simulink model "Demo_TISBeamShapes_cs"  (R2014b)
settings: Solver=FixedStepDiscrete  StartTime=0.0  StopTime=0.65  FixedStep=1/20  RelTol=1e-3
PreLoadFcn:
  | mbxruntime.callbacks.PreLoadFcn(bdroot);
  | check_NUTS_defined;
  | 
  | assignin('base',['model_closed_' bdroot],false);
PostLoadFcn:
  | mbxruntime.callbacks.PostLoadFcn(bdroot);
InitFcn:
  | mbxruntime.callbacks.InitFcn(bdroot);
StartFcn:
  | mbxruntime.callbacks.StartFcn(bdroot);
StopFcn:
  | mbxruntime.callbacks.StopFcn(bdroot);
model workspace: external: MAT-File (data not in the file)
undefined symbols (not defined in the file): Demo_TISBeamShapes_cs_011a8b437b9f8e69, Demo_TISBeamShapes_cs_0142ea2f1557d8d7, Demo_TISBeamShapes_cs_017a7d9bca76f440, Demo_TISBeamShapes_cs_024720c4bef5393b, Demo_TISBeamShapes_cs_02ccab9bad151289, Demo_TISBeamShapes_cs_0405f38d677d154d, Demo_TISBeamShapes_cs_04ff6bf95970c620, Demo_TISBeamShapes_cs_053dc575f3a51723, Demo_TISBeamShapes_cs_05aecbce86edff29, Demo_TISBeamShapes_cs_07e5aabef262ff79, Demo_TISBeamShapes_cs_09f6c52f0ff51ce9, Demo_TISBeamShapes_cs_0a8f57eb0b3b3045, Demo_TISBeamShapes_cs_0aa32373a6a68cd2, Demo_TISBeamShapes_cs_0afbbe5f5e24ce0f, Demo_TISBeamShapes_cs_0b39303de350ddcb, Demo_TISBeamShapes_cs_0b9be38c3822ef20, Demo_TISBeamShapes_cs_0c584d0ba0926c34, Demo_TISBeamShapes_cs_0d353a54ded74684, Demo_TISBeamShapes_cs_0e83e05019e43d52, Demo_TISBeamShapes_cs_0f04a582581737c0, Demo_TISBeamShapes_cs_1188b986555cf34f, Demo_TISBeamShapes_cs_11b8ea1198abf687, Demo_TISBeamShapes_cs_11c0571cd6471ba6, Demo_TISBeamShapes_cs_13caba5b40261316, Demo_TISBeamShapes_cs_15569a214ef5cb29, Demo_TISBeamShapes_cs_15f88ebb16dd7ea2, Demo_TISBeamShapes_cs_175a1fcf0f263ce1, Demo_TISBeamShapes_cs_1918ff8c81a32857, Demo_TISBeamShapes_cs_194e8e595a13d2e6, Demo_TISBeamShapes_cs_1a27a7dbb3fbcdbb, Demo_TISBeamShapes_cs_1a494c7f8641a573, Demo_TISBeamShapes_cs_1b017c38f43c5b4b, Demo_TISBeamShapes_cs_1c4cc580bee43225, Demo_TISBeamShapes_cs_1c9c39df8c9251aa, Demo_TISBeamShapes_cs_1d0978b5a4a81629, Demo_TISBeamShapes_cs_1f8d670963c68774, Demo_TISBeamShapes_cs_201dae5c2633ac72, Demo_TISBeamShapes_cs_204926faedc11b3b, Demo_TISBeamShapes_cs_207c04670db5631a, Demo_TISBeamShapes_cs_208dd3dde8789e89, Demo_TISBeamShapes_cs_20cecc5a76828476, Demo_TISBeamShapes_cs_20d64da55f57c800, Demo_TISBeamShapes_cs_21bd21ec0a5e9e24, Demo_TISBeamShapes_cs_21cca4ec9a0489e5, Demo_TISBeamShapes_cs_21d17805a232a810, Demo_TISBeamShapes_cs_22c7f73bd834d507, Demo_TISBeamShapes_cs_22e922ac5e27fa67, Demo_TISBeamShapes_cs_23a17c24d233256c, Demo_TISBeamShapes_cs_23d30f74b2f521d2, Demo_TISBeamShapes_cs_240dd111de20fa52, Demo_TISBeamShapes_cs_244be72567759b92, Demo_TISBeamShapes_cs_2541e0ae6c845c66, Demo_TISBeamShapes_cs_277df13a710d2e6d, Demo_TISBeamShapes_cs_278c9e9dccdcd54f, Demo_TISBeamShapes_cs_28fee81e926d7e28, Demo_TISBeamShapes_cs_29cd51f6b3d7013f, Demo_TISBeamShapes_cs_29d5b88c35ea84dd, Demo_TISBeamShapes_cs_29d910113b92e6ab, Demo_TISBeamShapes_cs_2a48985efc89fc6f, Demo_TISBeamShapes_cs_2b2ff84931628686 ... (+444)
libraries: PreScanSimulinkLibrary x168, PreScanUsefulBlocks x1
(part 1 of 27)
CloseFcn:
  | mbxruntime.callbacks.CloseFcn(bdroot);
  | evalin('base',['clear model_closed_' bdroot]);
settings Model: Creator=PRESCAN  LastModifiedBy=jenkins
settings DataIOCC: SignalLoggingSaveFormat=ModelDataLogs
settings OptimizationCC: InlineParams=on  ExpressionDepthLimit=2147483647  InitFltsAndDblsToZero=on
settings DebuggingCC: SaveWithParameterizedLinksMsg=none  UnderspecifiedInitializationDetection=Classic  MergeDetectMultiDrivingBlocksExec=none  SignalResolutionControl=TryResolveAllWithWarning  SolverPrmCheckMsg=none  MultiTaskDSMMsg=warning  MultiTaskCondExecSysMsg=none  FcnCallInpInsideContextMsg=UseLocalSettings  StateNameClashWarn=warning
settings ModelReferenceCC: UpdateModelReferenceTargets=IfOutOfDate
settings SFSimCC: SimParseCustomCode=off
settings SFSimCC: SimCustomHeaderCode=|
  | #include "prescan.h"
  | #include "prescan_platform.h"
settings RTWCC: IncludeERTFirstTime=on
settings GRTTargetCC: TargetFcnLib=ansi_tfl_tmw.mat  CombineOutputUpdateFcns=off  GRTInterface=on

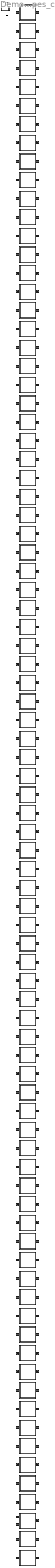
== system Demo_TISBeamShapes_cs ==
  note: Regenerate
  note: Simulink Mode
  note: Open Useful Blocks
  note: 2020.1.0
  note: Version:
  note: Author(s):
  note: N.A.
  note: Descriptive text:
  note: OBU-Beacon ID
  note: Demo Help
  note: This demo illustrates the use of the four possible beam shapes that are available for the TIS. It further illustrates how the TIS output is analyzed in Matlab. Keyword(s) - beamshape - beam - shape
  Cone_1 : Subsystem  Tag=WorldObjectSubSystem  InitFcn=UniqueId = '1098';
      mask init:
      | imagePath=which('Cone.jpg');
      mask Display: image(imread(imagePath));color('white');text(0, 0, ' ID=2\n')
  Controller : Subsystem  Description=8A3CD2955739A82C886C20AE3E253D78460D53180EE2C1B14CC08DF75A70BE77  Priority=-1  LoadFcn=load PreScanControllerData  mask(PreScan Simulation Controller){prescanversion='2020.1.0', ModelReferencing=off, TimeStep=1/20, ControlMode=0, PreScanExecutionMode=on, ControllerCount=0, ControllerIndex=0, ControllerOptions=''}
      mask prompts: prescanversion "PreScan Version"; ModelReferencing "Use Model Referencing"; TimeStep "Upload Period [s]"; ControlMode "Control Mode"; PreScanExecutionMode "Execution Mode"; ControllerCount "Controller Count"; ControllerIndex "Controller Index"; ControllerOptions "Controller Options"
      mask help: Please do not remove this block from the compilation sheet, as it connects the model to the PreScan environment.
      mask init:
      | model = bdroot(gcb);
      | ExperimentFile = mbxruntime.findExperimentFile(model,true); %relative path
      | 
      | [d1, d2, d3, prescandata] = prescan_Settings();
      | ModelDepo = fullfile(prescandata,'ModelDepo'); 
      | 
      | RTmode = mbxruntime.getRTMode(model);
      | 
      | SimulationMode = get_param(bdroot,'SimulationMode');
      | if strcmp(SimulationMode, 'rapid-accelerator')
      |     SimulationMode = 'external';
      | end
      | TargetName = get_param(bdroot,'SystemTargetFile');
      settings: ModelCloseFcn=assignin('base',['model_closed_' bdroot],true);
      mask Help: eval('openHelp(812)')
      mask Display: image(imread('prescanlogo.ico'))
  Cylinder_1 : Subsystem  Tag=WorldObjectSubSystem  InitFcn=UniqueId = '1102';
      mask init:
      | imagePath=which('Cylinder.jpg');
      mask Display: image(imread(imagePath));color('white');text(0, 0, ' ID=1\n')
  Cylinder_2 : Subsystem  Tag=WorldObjectSubSystem  InitFcn=UniqueId = '1103';
      mask init:
      | imagePath=which('Cylinder.jpg');
      mask Display: image(imread(imagePath));color('white');text(0, 0, ' ID=3\n')
  PreScanTerminator : Subsystem  Tag=PreScanTerminator  Priority=999  LoadFcn=load PrescanTerminatorData  mask(PreScan Simulation Terminator){TimeStep=1/20}
      mask prompts: TimeStep "Upload Period [s]"
      mask help: Please do not remove this block from the compilation sheet as it connects the model to the PreScan environment.
      mask Help: eval('openHelp(812)')
      mask Display: image(imread('prescanlogo.ico'))
  SELF_Cone_1 : Subsystem  Tag=sensor/SelfPort  Priority=30  LoadFcn=load('PreScanSelfSensorData.mat')  mask(PreScan Source Block: SELF){}
      mask help: The SELF port shows (state) information of the actor itself. The outputs are position in the experiment's axis system and the GPS coordinates, and the object's absolute velocity and compass heading. For more information, please click Help.
      settings: OpenFcn=open_system([gcb '/Sensor'],'mask')
      mask Help: eval('openHelp(462)')
      mask Display: image(imread('GPS.png'))
  SELF_Cylinder_1 : Subsystem  Tag=sensor/SelfPort  Priority=30  LoadFcn=load('PreScanSelfSensorData.mat')  mask(PreScan Source Block: SELF){}
      mask help: The SELF port shows (state) information of the actor itself. The outputs are position in the experiment's axis system and the GPS coordinates, and the object's absolute velocity and compass heading. For more information, please click Help.
      settings: OpenFcn=open_system([gcb '/Sensor'],'mask')
      mask Help: eval('openHelp(462)')
      mask Display: image(imread('GPS.png'))
  SELF_Cylinder_2 : Subsystem  Tag=sensor/SelfPort  Priority=30  LoadFcn=load('PreScanSelfSensorData.mat')  mask(PreScan Source Block: SELF){}
      mask help: The SELF port shows (state) information of the actor itself. The outputs are position in the experiment's axis system and the GPS coordinates, and the object's absolute velocity and compass heading. For more information, please click Help.
      settings: OpenFcn=open_system([gcb '/Sensor'],'mask')
      mask Help: eval('openHelp(462)')
      mask Display: image(imread('GPS.png'))
  SELF_Sphere_1 : Subsystem  Tag=sensor/SelfPort  Priority=30  LoadFcn=load('PreScanSelfSensorData.mat')  mask(PreScan Source Block: SELF){}
      mask help: The SELF port shows (state) information of the actor itself. The outputs are position in the experiment's axis system and the GPS coordinates, and the object's absolute velocity and compass heading. For more information, please click Help.
      settings: OpenFcn=open_system([gcb '/Sensor'],'mask')
      mask Help: eval('openHelp(462)')
      mask Display: image(imread('GPS.png'))
  SELF_Sphere_10 : Subsystem  Tag=sensor/SelfPort  Priority=30  LoadFcn=load('PreScanSelfSensorData.mat')  mask(PreScan Source Block: SELF){}
      mask help: The SELF port shows (state) information of the actor itself. The outputs are position in the experiment's axis system and the GPS coordinates, and the object's absolute velocity and compass heading. For more information, please click Help.
      settings: OpenFcn=open_system([gcb '/Sensor'],'mask')
      mask Help: eval('openHelp(462)')
      mask Display: image(imread('GPS.png'))
  SELF_Sphere_11 : Subsystem  Tag=sensor/SelfPort  Priority=30  LoadFcn=load('PreScanSelfSensorData.mat')  mask(PreScan Source Block: SELF){}
      mask help: The SELF port shows (state) information of the actor itself. The outputs are position in the experiment's axis system and the GPS coordinates, and the object's absolute velocity and compass heading. For more information, please click Help.
      settings: OpenFcn=open_system([gcb '/Sensor'],'mask')
      mask Help: eval('openHelp(462)')
      mask Display: image(imread('GPS.png'))
  SELF_Sphere_12 : Subsystem  Tag=sensor/SelfPort  Priority=30  LoadFcn=load('PreScanSelfSensorData.mat')  mask(PreScan Source Block: SELF){}
      mask help: The SELF port shows (state) information of the actor itself. The outputs are position in the experiment's axis system and the GPS coordinates, and the object's absolute velocity and compass heading. For more information, please click Help.
      settings: OpenFcn=open_system([gcb '/Sensor'],'mask')
      mask Help: eval('openHelp(462)')
      mask Display: image(imread('GPS.png'))
  SELF_Sphere_13 : Subsystem  Tag=sensor/SelfPort  Priority=30  LoadFcn=load('PreScanSelfSensorData.mat')  mask(PreScan Source Block: SELF){}
      mask help: The SELF port shows (state) information of the actor itself. The outputs are position in the experiment's axis system and the GPS coordinates, and the object's absolute velocity and compass heading. For more information, please click Help.
      settings: OpenFcn=open_system([gcb '/Sensor'],'mask')
      mask Help: eval('openHelp(462)')
      mask Display: image(imread('GPS.png'))
  SELF_Sphere_14 : Subsystem  Tag=sensor/SelfPort  Priority=30  LoadFcn=load('PreScanSelfSensorData.mat')  mask(PreScan Source Block: SELF){}
      mask help: The SELF port shows (state) information of the actor itself. The outputs are position in the experiment's axis system and the GPS coordinates, and the object's absolute velocity and compass heading. For more information, please click Help.
      settings: OpenFcn=open_system([gcb '/Sensor'],'mask')
      mask Help: eval('openHelp(462)')
      mask Display: image(imread('GPS.png'))
  SELF_Sphere_15 : Subsystem  Tag=sensor/SelfPort  Priority=30  LoadFcn=load('PreScanSelfSensorData.mat')  mask(PreScan Source Block: SELF){}
      mask help: The SELF port shows (state) information of the actor itself. The outputs are position in the experiment's axis system and the GPS coordinates, and the object's absolute velocity and compass heading. For more information, please click Help.
      settings: OpenFcn=open_system([gcb '/Sensor'],'mask')
      mask Help: eval('openHelp(462)')
      mask Display: image(imread('GPS.png'))
  SELF_Sphere_16 : Subsystem  Tag=sensor/SelfPort  Priority=30  LoadFcn=load('PreScanSelfSensorData.mat')  mask(PreScan Source Block: SELF){}
      mask help: The SELF port shows (state) information of the actor itself. The outputs are position in the experiment's axis system and the GPS coordinates, and the object's absolute velocity and compass heading. For more information, please click Help.
      settings: OpenFcn=open_system([gcb '/Sensor'],'mask')
      mask Help: eval('openHelp(462)')
      mask Display: image(imread('GPS.png'))
  SELF_Sphere_17 : Subsystem  Tag=sensor/SelfPort  Priority=30  LoadFcn=load('PreScanSelfSensorData.mat')  mask(PreScan Source Block: SELF){}
      mask help: The SELF port shows (state) information of the actor itself. The outputs are position in the experiment's axis system and the GPS coordinates, and the object's absolute velocity and compass heading. For more information, please click Help.
      settings: OpenFcn=open_system([gcb '/Sensor'],'mask')
      mask Help: eval('openHelp(462)')
      mask Display: image(imread('GPS.png'))
  SELF_Sphere_18 : Subsystem  Tag=sensor/SelfPort  Priority=30  LoadFcn=load('PreScanSelfSensorData.mat')  mask(PreScan Source Block: SELF){}
      mask help: The SELF port shows (state) information of the actor itself. The outputs are position in the experiment's axis system and the GPS coordinates, and the object's absolute velocity and compass heading. For more information, please click Help.
      settings: OpenFcn=open_system([gcb '/Sensor'],'mask')
      mask Help: eval('openHelp(462)')
      mask Display: image(imread('GPS.png'))
  SELF_Sphere_19 : Subsystem  Tag=sensor/SelfPort  Priority=30  LoadFcn=load('PreScanSelfSensorData.mat')  mask(PreScan Source Block: SELF){}
      mask help: The SELF port shows (state) information of the actor itself. The outputs are position in the experiment's axis system and the GPS coordinates, and the object's absolute velocity and compass heading. For more information, please click Help.
      settings: OpenFcn=open_system([gcb '/Sensor'],'mask')
      mask Help: eval('openHelp(462)')
      mask Display: image(imread('GPS.png'))
  SELF_Sphere_2 : Subsystem  Tag=sensor/SelfPort  Priority=30  LoadFcn=load('PreScanSelfSensorData.mat')  mask(PreScan Source Block: SELF){}
      mask help: The SELF port shows (state) information of the actor itself. The outputs are position in the experiment's axis system and the GPS coordinates, and the object's absolute velocity and compass heading. For more information, please click Help.
      settings: OpenFcn=open_system([gcb '/Sensor'],'mask')
      mask Help: eval('openHelp(462)')
      mask Display: image(imread('GPS.png'))
  SELF_Sphere_20 : Subsystem  Tag=sensor/SelfPort  Priority=30  LoadFcn=load('PreScanSelfSensorData.mat')  mask(PreScan Source Block: SELF){}
      mask help: The SELF port shows (state) information of the actor itself. The outputs are position in the experiment's axis system and the GPS coordinates, and the object's absolute velocity and compass heading. For more information, please click Help.
      settings: OpenFcn=open_system([gcb '/Sensor'],'mask')
      mask Help: eval('openHelp(462)')
      mask Display: image(imread('GPS.png'))
  SELF_Sphere_21 : Subsystem  Tag=sensor/SelfPort  Priority=30  LoadFcn=load('PreScanSelfSensorData.mat')  mask(PreScan Source Block: SELF){}
      mask help: The SELF port shows (state) information of the actor itself. The outputs are position in the experiment's axis system and the GPS coordinates, and the object's absolute velocity and compass heading. For more information, please click Help.
      settings: OpenFcn=open_system([gcb '/Sensor'],'mask')
      mask Help: eval('openHelp(462)')
      mask Display: image(imread('GPS.png'))
  SELF_Sphere_22 : Subsystem  Tag=sensor/SelfPort  Priority=30  LoadFcn=load('PreScanSelfSensorData.mat')  mask(PreScan Source Block: SELF){}
      mask help: The SELF port shows (state) information of the actor itself. The outputs are position in the experiment's axis system and the GPS coordinates, and the object's absolute velocity and compass heading. For more information, please click Help.
      settings: OpenFcn=open_system([gcb '/Sensor'],'mask')
      mask Help: eval('openHelp(462)')
      mask Display: image(imread('GPS.png'))
  SELF_Sphere_23 : Subsystem  Tag=sensor/SelfPort  Priority=30  LoadFcn=load('PreScanSelfSensorData.mat')  mask(PreScan Source Block: SELF){}
      mask help: The SELF port shows (state) information of the actor itself. The outputs are position in the experiment's axis system and the GPS coordinates, and the object's absolute velocity and compass heading. For more information, please click Help.
      settings: OpenFcn=open_system([gcb '/Sensor'],'mask')
      mask Help: eval('openHelp(462)')
      mask Display: image(imread('GPS.png'))
  SELF_Sphere_24 : Subsystem  Tag=sensor/SelfPort  Priority=30  LoadFcn=load('PreScanSelfSensorData.mat')  mask(PreScan Source Block: SELF){}
      mask help: The SELF port shows (state) information of the actor itself. The outputs are position in the experiment's axis system and the GPS coordinates, and the object's absolute velocity and compass heading. For more information, please click Help.
      settings: OpenFcn=open_system([gcb '/Sensor'],'mask')
      mask Help: eval('openHelp(462)')
      mask Display: image(imread('GPS.png'))
  SELF_Sphere_25 : Subsystem  Tag=sensor/SelfPort  Priority=30  LoadFcn=load('PreScanSelfSensorData.mat')  mask(PreScan Source Block: SELF){}
      mask help: The SELF port shows (state) information of the actor itself. The outputs are position in the experiment's axis system and the GPS coordinates, and the object's absolute velocity and compass heading. For more information, please click Help.
      settings: OpenFcn=open_system([gcb '/Sensor'],'mask')
      mask Help: eval('openHelp(462)')
      mask Display: image(imread('GPS.png'))
  SELF_Sphere_26 : Subsystem  Tag=sensor/SelfPort  Priority=30  LoadFcn=load('PreScanSelfSensorData.mat')  mask(PreScan Source Block: SELF){}
      mask help: The SELF port shows (state) information of the actor itself. The outputs are position in the experiment's axis system and the GPS coordinates, and the object's absolute velocity and compass heading. For more information, please click Help.
      settings: OpenFcn=open_system([gcb '/Sensor'],'mask')
      mask Help: eval('openHelp(462)')
      mask Display: image(imread('GPS.png'))
  SELF_Sphere_27 : Subsystem  Tag=sensor/SelfPort  Priority=30  LoadFcn=load('PreScanSelfSensorData.mat')  mask(PreScan Source Block: SELF){}
      mask help: The SELF port shows (state) information of the actor itself. The outputs are position in the experiment's axis system and the GPS coordinates, and the object's absolute velocity and compass heading. For more information, please click Help.
      settings: OpenFcn=open_system([gcb '/Sensor'],'mask')
      mask Help: eval('openHelp(462)')
      mask Display: image(imread('GPS.png'))
  SELF_Sphere_28 : Subsystem  Tag=sensor/SelfPort  Priority=30  LoadFcn=load('PreScanSelfSensorData.mat')  mask(PreScan Source Block: SELF){}
      mask help: The SELF port shows (state) information of the actor itself. The outputs are position in the experiment's axis system and the GPS coordinates, and the object's absolute velocity and compass heading. For more information, please click Help.
      settings: OpenFcn=open_system([gcb '/Sensor'],'mask')
      mask Help: eval('openHelp(462)')
      mask Display: image(imread('GPS.png'))
  SELF_Sphere_29 : Subsystem  Tag=sensor/SelfPort  Priority=30  LoadFcn=load('PreScanSelfSensorData.mat')  mask(PreScan Source Block: SELF){}
      mask help: The SELF port shows (state) information of the actor itself. The outputs are position in the experiment's axis system and the GPS coordinates, and the object's absolute velocity and compass heading. For more information, please click Help.
      settings: OpenFcn=open_system([gcb '/Sensor'],'mask')
      mask Help: eval('openHelp(462)')
      mask Display: image(imread('GPS.png'))
  SELF_Sphere_3 : Subsystem  Tag=sensor/SelfPort  Priority=30  LoadFcn=load('PreScanSelfSensorData.mat')  mask(PreScan Source Block: SELF){}
      mask help: The SELF port shows (state) information of the actor itself. The outputs are position in the experiment's axis system and the GPS coordinates, and the object's absolute velocity and compass heading. For more information, please click Help.
      settings: OpenFcn=open_system([gcb '/Sensor'],'mask')
      mask Help: eval('openHelp(462)')
      mask Display: image(imread('GPS.png'))
  SELF_Sphere_30 : Subsystem  Tag=sensor/SelfPort  Priority=30  LoadFcn=load('PreScanSelfSensorData.mat')  mask(PreScan Source Block: SELF){}
      mask help: The SELF port shows (state) information of the actor itself. The outputs are position in the experiment's axis system and the GPS coordinates, and the object's absolute velocity and compass heading. For more information, please click Help.
      settings: OpenFcn=open_system([gcb '/Sensor'],'mask')
      mask Help: eval('openHelp(462)')
      mask Display: image(imread('GPS.png'))
  SELF_Sphere_31 : Subsystem  Tag=sensor/SelfPort  Priority=30  LoadFcn=load('PreScanSelfSensorData.mat')  mask(PreScan Source Block: SELF){}
      mask help: The SELF port shows (state) information of the actor itself. The outputs are position in the experiment's axis system and the GPS coordinates, and the object's absolute velocity and compass heading. For more information, please click Help.
      settings: OpenFcn=open_system([gcb '/Sensor'],'mask')
      mask Help: eval('openHelp(462)')
      mask Display: image(imread('GPS.png'))
  SELF_Sphere_32 : Subsystem  Tag=sensor/SelfPort  Priority=30  LoadFcn=load('PreScanSelfSensorData.mat')  mask(PreScan Source Block: SELF){}
      mask help: The SELF port shows (state) information of the actor itself. The outputs are position in the experiment's axis system and the GPS coordinates, and the object's absolute velocity and compass heading. For more information, please click Help.
      settings: OpenFcn=open_system([gcb '/Sensor'],'mask')
      mask Help: eval('openHelp(462)')
      mask Display: image(imread('GPS.png'))
  SELF_Sphere_33 : Subsystem  Tag=sensor/SelfPort  Priority=30  LoadFcn=load('PreScanSelfSensorData.mat')  mask(PreScan Source Block: SELF){}
      mask help: The SELF port shows (state) information of the actor itself. The outputs are position in the experiment's axis system and the GPS coordinates, and the object's absolute velocity and compass heading. For more information, please click Help.
      settings: OpenFcn=open_system([gcb '/Sensor'],'mask')
      mask Help: eval('openHelp(462)')
      mask Display: image(imread('GPS.png'))
  SELF_Sphere_34 : Subsystem  Tag=sensor/SelfPort  Priority=30  LoadFcn=load('PreScanSelfSensorData.mat')  mask(PreScan Source Block: SELF){}
      mask help: The SELF port shows (state) information of the actor itself. The outputs are position in the experiment's axis system and the GPS coordinates, and the object's absolute velocity and compass heading. For more information, please click Help.
      settings: OpenFcn=open_system([gcb '/Sensor'],'mask')
      mask Help: eval('openHelp(462)')
      mask Display: image(imread('GPS.png'))
  SELF_Sphere_35 : Subsystem  Tag=sensor/SelfPort  Priority=30  LoadFcn=load('PreScanSelfSensorData.mat')  mask(PreScan Source Block: SELF){}
      mask help: The SELF port shows (state) information of the actor itself. The outputs are position in the experiment's axis system and the GPS coordinates, and the object's absolute velocity and compass heading. For more information, please click Help.
      settings: OpenFcn=open_system([gcb '/Sensor'],'mask')
      mask Help: eval('openHelp(462)')
      mask Display: image(imread('GPS.png'))
  SELF_Sphere_36 : Subsystem  Tag=sensor/SelfPort  Priority=30  LoadFcn=load('PreScanSelfSensorData.mat')  mask(PreScan Source Block: SELF){}
      mask help: The SELF port shows (state) information of the actor itself. The outputs are position in the experiment's axis system and the GPS coordinates, and the object's absolute velocity and compass heading. For more information, please click Help.
      settings: OpenFcn=open_system([gcb '/Sensor'],'mask')
      mask Help: eval('openHelp(462)')
      mask Display: image(imread('GPS.png'))
  SELF_Sphere_37 : Subsystem  Tag=sensor/SelfPort  Priority=30  LoadFcn=load('PreScanSelfSensorData.mat')  mask(PreScan Source Block: SELF){}
      mask help: The SELF port shows (state) information of the actor itself. The outputs are position in the experiment's axis system and the GPS coordinates, and the object's absolute velocity and compass heading. For more information, please click Help.
      settings: OpenFcn=open_system([gcb '/Sensor'],'mask')
      mask Help: eval('openHelp(462)')
      mask Display: image(imread('GPS.png'))
  SELF_Sphere_38 : Subsystem  Tag=sensor/SelfPort  Priority=30  LoadFcn=load('PreScanSelfSensorData.mat')  mask(PreScan Source Block: SELF){}
      mask help: The SELF port shows (state) information of the actor itself. The outputs are position in the experiment's axis system and the GPS coordinates, and the object's absolute velocity and compass heading. For more information, please click Help.
      settings: OpenFcn=open_system([gcb '/Sensor'],'mask')
      mask Help: eval('openHelp(462)')
      mask Display: image(imread('GPS.png'))
  SELF_Sphere_39 : Subsystem  Tag=sensor/SelfPort  Priority=30  LoadFcn=load('PreScanSelfSensorData.mat')  mask(PreScan Source Block: SELF){}
      mask help: The SELF port shows (state) information of the actor itself. The outputs are position in the experiment's axis system and the GPS coordinates, and the object's absolute velocity and compass heading. For more information, please click Help.
      settings: OpenFcn=open_system([gcb '/Sensor'],'mask')
      mask Help: eval('openHelp(462)')
      mask Display: image(imread('GPS.png'))
  SELF_Sphere_4 : Subsystem  Tag=sensor/SelfPort  Priority=30  LoadFcn=load('PreScanSelfSensorData.mat')  mask(PreScan Source Block: SELF){}
      mask help: The SELF port shows (state) information of the actor itself. The outputs are position in the experiment's axis system and the GPS coordinates, and the object's absolute velocity and compass heading. For more information, please click Help.
      settings: OpenFcn=open_system([gcb '/Sensor'],'mask')
      mask Help: eval('openHelp(462)')
      mask Display: image(imread('GPS.png'))
  SELF_Sphere_40 : Subsystem  Tag=sensor/SelfPort  Priority=30  LoadFcn=load('PreScanSelfSensorData.mat')  mask(PreScan Source Block: SELF){}
      mask help: The SELF port shows (state) information of the actor itself. The outputs are position in the experiment's axis system and the GPS coordinates, and the object's absolute velocity and compass heading. For more information, please click Help.
      settings: OpenFcn=open_system([gcb '/Sensor'],'mask')
      mask Help: eval('openHelp(462)')
      mask Display: image(imread('GPS.png'))
  SELF_Sphere_41 : Subsystem  Tag=sensor/SelfPort  Priority=30  LoadFcn=load('PreScanSelfSensorData.mat')  mask(PreScan Source Block: SELF){}
      mask help: The SELF port shows (state) information of the actor itself. The outputs are position in the experiment's axis system and the GPS coordinates, and the object's absolute velocity and compass heading. For more information, please click Help.
      settings: OpenFcn=open_system([gcb '/Sensor'],'mask')
      mask Help: eval('openHelp(462)')
      mask Display: image(imread('GPS.png'))
  SELF_Sphere_42 : Subsystem  Tag=sensor/SelfPort  Priority=30  LoadFcn=load('PreScanSelfSensorData.mat')  mask(PreScan Source Block: SELF){}
      mask help: The SELF port shows (state) information of the actor itself. The outputs are position in the experiment's axis system and the GPS coordinates, and the object's absolute velocity and compass heading. For more information, please click Help.
      settings: OpenFcn=open_system([gcb '/Sensor'],'mask')
      mask Help: eval('openHelp(462)')
      mask Display: image(imread('GPS.png'))
  SELF_Sphere_43 : Subsystem  Tag=sensor/SelfPort  Priority=30  LoadFcn=load('PreScanSelfSensorData.mat')  mask(PreScan Source Block: SELF){}
      mask help: The SELF port shows (state) information of the actor itself. The outputs are position in the experiment's axis system and the GPS coordinates, and the object's absolute velocity and compass heading. For more information, please click Help.
      settings: OpenFcn=open_system([gcb '/Sensor'],'mask')
      mask Help: eval('openHelp(462)')
      mask Display: image(imread('GPS.png'))
  SELF_Sphere_44 : Subsystem  Tag=sensor/SelfPort  Priority=30  LoadFcn=load('PreScanSelfSensorData.mat')  mask(PreScan Source Block: SELF){}
      mask help: The SELF port shows (state) information of the actor itself. The outputs are position in the experiment's axis system and the GPS coordinates, and the object's absolute velocity and compass heading. For more information, please click Help.
      settings: OpenFcn=open_system([gcb '/Sensor'],'mask')
      mask Help: eval('openHelp(462)')
      mask Display: image(imread('GPS.png'))
  SELF_Sphere_45 : Subsystem  Tag=sensor/SelfPort  Priority=30  LoadFcn=load('PreScanSelfSensorData.mat')  mask(PreScan Source Block: SELF){}
      mask help: The SELF port shows (state) information of the actor itself. The outputs are position in the experiment's axis system and the GPS coordinates, and the object's absolute velocity and compass heading. For more information, please click Help.
      settings: OpenFcn=open_system([gcb '/Sensor'],'mask')
      mask Help: eval('openHelp(462)')
      mask Display: image(imread('GPS.png'))
  SELF_Sphere_46 : Subsystem  Tag=sensor/SelfPort  Priority=30  LoadFcn=load('PreScanSelfSensorData.mat')  mask(PreScan Source Block: SELF){}
      mask help: The SELF port shows (state) information of the actor itself. The outputs are position in the experiment's axis system and the GPS coordinates, and the object's absolute velocity and compass heading. For more information, please click Help.
      settings: OpenFcn=open_system([gcb '/Sensor'],'mask')
      mask Help: eval('openHelp(462)')
      mask Display: image(imread('GPS.png'))
  SELF_Sphere_47 : Subsystem  Tag=sensor/SelfPort  Priority=30  LoadFcn=load('PreScanSelfSensorData.mat')  mask(PreScan Source Block: SELF){}
      mask help: The SELF port shows (state) information of the actor itself. The outputs are position in the experiment's axis system and the GPS coordinates, and the object's absolute velocity and compass heading. For more information, please click Help.
      settings: OpenFcn=open_system([gcb '/Sensor'],'mask')
      mask Help: eval('openHelp(462)')
      mask Display: image(imread('GPS.png'))
  SELF_Sphere_48 : Subsystem  Tag=sensor/SelfPort  Priority=30  LoadFcn=load('PreScanSelfSensorData.mat')  mask(PreScan Source Block: SELF){}
      mask help: The SELF port shows (state) information of the actor itself. The outputs are position in the experiment's axis system and the GPS coordinates, and the object's absolute velocity and compass heading. For more information, please click Help.
      settings: OpenFcn=open_system([gcb '/Sensor'],'mask')
      mask Help: eval('openHelp(462)')
      mask Display: image(imread('GPS.png'))
  SELF_Sphere_49 : Subsystem  Tag=sensor/SelfPort  Priority=30  LoadFcn=load('PreScanSelfSensorData.mat')  mask(PreScan Source Block: SELF){}
      mask help: The SELF port shows (state) information of the actor itself. The outputs are position in the experiment's axis system and the GPS coordinates, and the object's absolute velocity and compass heading. For more information, please click Help.
      settings: OpenFcn=open_system([gcb '/Sensor'],'mask')
      mask Help: eval('openHelp(462)')
      mask Display: image(imread('GPS.png'))
  SELF_Sphere_5 : Subsystem  Tag=sensor/SelfPort  Priority=30  LoadFcn=load('PreScanSelfSensorData.mat')  mask(PreScan Source Block: SELF){}
      mask help: The SELF port shows (state) information of the actor itself. The outputs are position in the experiment's axis system and the GPS coordinates, and the object's absolute velocity and compass heading. For more information, please click Help.
      settings: OpenFcn=open_system([gcb '/Sensor'],'mask')
      mask Help: eval('openHelp(462)')
      mask Display: image(imread('GPS.png'))
  SELF_Sphere_50 : Subsystem  Tag=sensor/SelfPort  Priority=30  LoadFcn=load('PreScanSelfSensorData.mat')  mask(PreScan Source Block: SELF){}
      mask help: The SELF port shows (state) information of the actor itself. The outputs are position in the experiment's axis system and the GPS coordinates, and the object's absolute velocity and compass heading. For more information, please click Help.
      settings: OpenFcn=open_system([gcb '/Sensor'],'mask')
      mask Help: eval('openHelp(462)')
      mask Display: image(imread('GPS.png'))
  SELF_Sphere_51 : Subsystem  Tag=sensor/SelfPort  Priority=30  LoadFcn=load('PreScanSelfSensorData.mat')  mask(PreScan Source Block: SELF){}
      mask help: The SELF port shows (state) information of the actor itself. The outputs are position in the experiment's axis system and the GPS coordinates, and the object's absolute velocity and compass heading. For more information, please click Help.
      settings: OpenFcn=open_system([gcb '/Sensor'],'mask')
      mask Help: eval('openHelp(462)')
      mask Display: image(imread('GPS.png'))
  SELF_Sphere_52 : Subsystem  Tag=sensor/SelfPort  Priority=30  LoadFcn=load('PreScanSelfSensorData.mat')  mask(PreScan Source Block: SELF){}
      mask help: The SELF port shows (state) information of the actor itself. The outputs are position in the experiment's axis system and the GPS coordinates, and the object's absolute velocity and compass heading. For more information, please click Help.
      settings: OpenFcn=open_system([gcb '/Sensor'],'mask')
      mask Help: eval('openHelp(462)')
      mask Display: image(imread('GPS.png'))
  SELF_Sphere_53 : Subsystem  Tag=sensor/SelfPort  Priority=30  LoadFcn=load('PreScanSelfSensorData.mat')  mask(PreScan Source Block: SELF){}
      mask help: The SELF port shows (state) information of the actor itself. The outputs are position in the experiment's axis system and the GPS coordinates, and the object's absolute velocity and compass heading. For more information, please click Help.
      settings: OpenFcn=open_system([gcb '/Sensor'],'mask')
      mask Help: eval('openHelp(462)')
      mask Display: image(imread('GPS.png'))
  SELF_Sphere_54 : Subsystem  Tag=sensor/SelfPort  Priority=30  LoadFcn=load('PreScanSelfSensorData.mat')  mask(PreScan Source Block: SELF){}
      mask help: The SELF port shows (state) information of the actor itself. The outputs are position in the experiment's axis system and the GPS coordinates, and the object's absolute velocity and compass heading. For more information, please click Help.
      settings: OpenFcn=open_system([gcb '/Sensor'],'mask')
      mask Help: eval('openHelp(462)')
      mask Display: image(imread('GPS.png'))
  SELF_Sphere_55 : Subsystem  Tag=sensor/SelfPort  Priority=30  LoadFcn=load('PreScanSelfSensorData.mat')  mask(PreScan Source Block: SELF){}
      mask help: The SELF port shows (state) information of the actor itself. The outputs are position in the experiment's axis system and the GPS coordinates, and the object's absolute velocity and compass heading. For more information, please click Help.
      settings: OpenFcn=open_system([gcb '/Sensor'],'mask')
      mask Help: eval('openHelp(462)')
      mask Display: image(imread('GPS.png'))
  SELF_Sphere_56 : Subsystem  Tag=sensor/SelfPort  Priority=30  LoadFcn=load('PreScanSelfSensorData.mat')  mask(PreScan Source Block: SELF){}
      mask help: The SELF port shows (state) information of the actor itself. The outputs are position in the experiment's axis system and the GPS coordinates, and the object's absolute velocity and compass heading. For more information, please click Help.
      settings: OpenFcn=open_system([gcb '/Sensor'],'mask')
      mask Help: eval('openHelp(462)')
      mask Display: image(imread('GPS.png'))
  SELF_Sphere_57 : Subsystem  Tag=sensor/SelfPort  Priority=30  LoadFcn=load('PreScanSelfSensorData.mat')  mask(PreScan Source Block: SELF){}
      mask help: The SELF port shows (state) information of the actor itself. The outputs are position in the experiment's axis system and the GPS coordinates, and the object's absolute velocity and compass heading. For more information, please click Help.
      settings: OpenFcn=open_system([gcb '/Sensor'],'mask')
      mask Help: eval('openHelp(462)')
      mask Display: image(imread('GPS.png'))
  SELF_Sphere_58 : Subsystem  Tag=sensor/SelfPort  Priority=30  LoadFcn=load('PreScanSelfSensorData.mat')  mask(PreScan Source Block: SELF){}
      mask help: The SELF port shows (state) information of the actor itself. The outputs are position in the experiment's axis system and the GPS coordinates, and the object's absolute velocity and compass heading. For more information, please click Help.
      settings: OpenFcn=open_system([gcb '/Sensor'],'mask')
      mask Help: eval('openHelp(462)')
      mask Display: image(imread('GPS.png'))
  SELF_Sphere_59 : Subsystem  Tag=sensor/SelfPort  Priority=30  LoadFcn=load('PreScanSelfSensorData.mat')  mask(PreScan Source Block: SELF){}
      mask help: The SELF port shows (state) information of the actor itself. The outputs are position in the experiment's axis system and the GPS coordinates, and the object's absolute velocity and compass heading. For more information, please click Help.
      settings: OpenFcn=open_system([gcb '/Sensor'],'mask')
      mask Help: eval('openHelp(462)')
      mask Display: image(imread('GPS.png'))
  SELF_Sphere_6 : Subsystem  Tag=sensor/SelfPort  Priority=30  LoadFcn=load('PreScanSelfSensorData.mat')  mask(PreScan Source Block: SELF){}
      mask help: The SELF port shows (state) information of the actor itself. The outputs are position in the experiment's axis system and the GPS coordinates, and the object's absolute velocity and compass heading. For more information, please click Help.
      settings: OpenFcn=open_system([gcb '/Sensor'],'mask')
      mask Help: eval('openHelp(462)')
      mask Display: image(imread('GPS.png'))
  SELF_Sphere_60 : Subsystem  Tag=sensor/SelfPort  Priority=30  LoadFcn=load('PreScanSelfSensorData.mat')  mask(PreScan Source Block: SELF){}
      mask help: The SELF port shows (state) information of the actor itself. The outputs are position in the experiment's axis system and the GPS coordinates, and the object's absolute velocity and compass heading. For more information, please click Help.
      settings: OpenFcn=open_system([gcb '/Sensor'],'mask')
      mask Help: eval('openHelp(462)')
      mask Display: image(imread('GPS.png'))
  SELF_Sphere_61 : Subsystem  Tag=sensor/SelfPort  Priority=30  LoadFcn=load('PreScanSelfSensorData.mat')  mask(PreScan Source Block: SELF){}
      mask help: The SELF port shows (state) information of the actor itself. The outputs are position in the experiment's axis system and the GPS coordinates, and the object's absolute velocity and compass heading. For more information, please click Help.
      settings: OpenFcn=open_system([gcb '/Sensor'],'mask')
      mask Help: eval('openHelp(462)')
      mask Display: image(imread('GPS.png'))
  SELF_Sphere_62 : Subsystem  Tag=sensor/SelfPort  Priority=30  LoadFcn=load('PreScanSelfSensorData.mat')  mask(PreScan Source Block: SELF){}
      mask help: The SELF port shows (state) information of the actor itself. The outputs are position in the experiment's axis system and the GPS coordinates, and the object's absolute velocity and compass heading. For more information, please click Help.
      settings: OpenFcn=open_system([gcb '/Sensor'],'mask')
      mask Help: eval('openHelp(462)')
      mask Display: image(imread('GPS.png'))
  SELF_Sphere_63 : Subsystem  Tag=sensor/SelfPort  Priority=30  LoadFcn=load('PreScanSelfSensorData.mat')  mask(PreScan Source Block: SELF){}
      mask help: The SELF port shows (state) information of the actor itself. The outputs are position in the experiment's axis system and the GPS coordinates, and the object's absolute velocity and compass heading. For more information, please click Help.
      settings: OpenFcn=open_system([gcb '/Sensor'],'mask')
      mask Help: eval('openHelp(462)')
      mask Display: image(imread('GPS.png'))
  SELF_Sphere_64 : Subsystem  Tag=sensor/SelfPort  Priority=30  LoadFcn=load('PreScanSelfSensorData.mat')  mask(PreScan Source Block: SELF){}
      mask help: The SELF port shows (state) information of the actor itself. The outputs are position in the experiment's axis system and the GPS coordinates, and the object's absolute velocity and compass heading. For more information, please click Help.
      settings: OpenFcn=open_system([gcb '/Sensor'],'mask')
      mask Help: eval('openHelp(462)')
      mask Display: image(imread('GPS.png'))
  SELF_Sphere_65 : Subsystem  Tag=sensor/SelfPort  Priority=30  LoadFcn=load('PreScanSelfSensorData.mat')  mask(PreScan Source Block: SELF){}
      mask help: The SELF port shows (state) information of the actor itself. The outputs are position in the experiment's axis system and the GPS coordinates, and the object's absolute velocity and compass heading. For more information, please click Help.
      settings: OpenFcn=open_system([gcb '/Sensor'],'mask')
      mask Help: eval('openHelp(462)')
      mask Display: image(imread('GPS.png'))
  SELF_Sphere_66 : Subsystem  Tag=sensor/SelfPort  Priority=30  LoadFcn=load('PreScanSelfSensorData.mat')  mask(PreScan Source Block: SELF){}
      mask help: The SELF port shows (state) information of the actor itself. The outputs are position in the experiment's axis system and the GPS coordinates, and the object's absolute velocity and compass heading. For more information, please click Help.
      settings: OpenFcn=open_system([gcb '/Sensor'],'mask')
      mask Help: eval('openHelp(462)')
      mask Display: image(imread('GPS.png'))
  SELF_Sphere_67 : Subsystem  Tag=sensor/SelfPort  Priority=30  LoadFcn=load('PreScanSelfSensorData.mat')  mask(PreScan Source Block: SELF){}
      mask help: The SELF port shows (state) information of the actor itself. The outputs are position in the experiment's axis system and the GPS coordinates, and the object's absolute velocity and compass heading. For more information, please click Help.
      settings: OpenFcn=open_system([gcb '/Sensor'],'mask')
      mask Help: eval('openHelp(462)')
      mask Display: image(imread('GPS.png'))
  SELF_Sphere_68 : Subsystem  Tag=sensor/SelfPort  Priority=30  LoadFcn=load('PreScanSelfSensorData.mat')  mask(PreScan Source Block: SELF){}
      mask help: The SELF port shows (state) information of the actor itself. The outputs are position in the experiment's axis system and the GPS coordinates, and the object's absolute velocity and compass heading. For more information, please click Help.
      settings: OpenFcn=open_system([gcb '/Sensor'],'mask')
      mask Help: eval('openHelp(462)')
      mask Display: image(imread('GPS.png'))
  SELF_Sphere_69 : Subsystem  Tag=sensor/SelfPort  Priority=30  LoadFcn=load('PreScanSelfSensorData.mat')  mask(PreScan Source Block: SELF){}
      mask help: The SELF port shows (state) information of the actor itself. The outputs are position in the experiment's axis system and the GPS coordinates, and the object's absolute velocity and compass heading. For more information, please click Help.
      settings: OpenFcn=open_system([gcb '/Sensor'],'mask')
      mask Help: eval('openHelp(462)')
      mask Display: image(imread('GPS.png'))
  SELF_Sphere_7 : Subsystem  Tag=sensor/SelfPort  Priority=30  LoadFcn=load('PreScanSelfSensorData.mat')  mask(PreScan Source Block: SELF){}
      mask help: The SELF port shows (state) information of the actor itself. The outputs are position in the experiment's axis system and the GPS coordinates, and the object's absolute velocity and compass heading. For more information, please click Help.
      settings: OpenFcn=open_system([gcb '/Sensor'],'mask')
      mask Help: eval('openHelp(462)')
      mask Display: image(imread('GPS.png'))
  SELF_Sphere_70 : Subsystem  Tag=sensor/SelfPort  Priority=30  LoadFcn=load('PreScanSelfSensorData.mat')  mask(PreScan Source Block: SELF){}
      mask help: The SELF port shows (state) information of the actor itself. The outputs are position in the experiment's axis system and the GPS coordinates, and the object's absolute velocity and compass heading. For more information, please click Help.
      settings: OpenFcn=open_system([gcb '/Sensor'],'mask')
      mask Help: eval('openHelp(462)')
      mask Display: image(imread('GPS.png'))
  SELF_Sphere_71 : Subsystem  Tag=sensor/SelfPort  Priority=30  LoadFcn=load('PreScanSelfSensorData.mat')  mask(PreScan Source Block: SELF){}
      mask help: The SELF port shows (state) information of the actor itself. The outputs are position in the experiment's axis system and the GPS coordinates, and the object's absolute velocity and compass heading. For more information, please click Help.
      settings: OpenFcn=open_system([gcb '/Sensor'],'mask')
      mask Help: eval('openHelp(462)')
      mask Display: image(imread('GPS.png'))
  SELF_Sphere_72 : Subsystem  Tag=sensor/SelfPort  Priority=30  LoadFcn=load('PreScanSelfSensorData.mat')  mask(PreScan Source Block: SELF){}
      mask help: The SELF port shows (state) information of the actor itself. The outputs are position in the experiment's axis system and the GPS coordinates, and the object's absolute velocity and compass heading. For more information, please click Help.
      settings: OpenFcn=open_system([gcb '/Sensor'],'mask')
      mask Help: eval('openHelp(462)')
      mask Display: image(imread('GPS.png'))
  SELF_Sphere_73 : Subsystem  Tag=sensor/SelfPort  Priority=30  LoadFcn=load('PreScanSelfSensorData.mat')  mask(PreScan Source Block: SELF){}
      mask help: The SELF port shows (state) information of the actor itself. The outputs are position in the experiment's axis system and the GPS coordinates, and the object's absolute velocity and compass heading. For more information, please click Help.
      settings: OpenFcn=open_system([gcb '/Sensor'],'mask')
      mask Help: eval('openHelp(462)')
      mask Display: image(imread('GPS.png'))
  SELF_Sphere_74 : Subsystem  Tag=sensor/SelfPort  Priority=30  LoadFcn=load('PreScanSelfSensorData.mat')  mask(PreScan Source Block: SELF){}
      mask help: The SELF port shows (state) information of the actor itself. The outputs are position in the experiment's axis system and the GPS coordinates, and the object's absolute velocity and compass heading. For more information, please click Help.
      settings: OpenFcn=open_system([gcb '/Sensor'],'mask')
      mask Help: eval('openHelp(462)')
      mask Display: image(imread('GPS.png'))
  SELF_Sphere_75 : Subsystem  Tag=sensor/SelfPort  Priority=30  LoadFcn=load('PreScanSelfSensorData.mat')  mask(PreScan Source Block: SELF){}
      mask help: The SELF port shows (state) information of the actor itself. The outputs are position in the experiment's axis system and the GPS coordinates, and the object's absolute velocity and compass heading. For more information, please click Help.
      settings: OpenFcn=open_system([gcb '/Sensor'],'mask')
      mask Help: eval('openHelp(462)')
      mask Display: image(imread('GPS.png'))
  SELF_Sphere_76 : Subsystem  Tag=sensor/SelfPort  Priority=30  LoadFcn=load('PreScanSelfSensorData.mat')  mask(PreScan Source Block: SELF){}
      mask help: The SELF port shows (state) information of the actor itself. The outputs are position in the experiment's axis system and the GPS coordinates, and the object's absolute velocity and compass heading. For more information, please click Help.
      settings: OpenFcn=open_system([gcb '/Sensor'],'mask')
      mask Help: eval('openHelp(462)')
      mask Display: image(imread('GPS.png'))
  SELF_Sphere_77 : Subsystem  Tag=sensor/SelfPort  Priority=30  LoadFcn=load('PreScanSelfSensorData.mat')  mask(PreScan Source Block: SELF){}
      mask help: The SELF port shows (state) information of the actor itself. The outputs are position in the experiment's axis system and the GPS coordinates, and the object's absolute velocity and compass heading. For more information, please click Help.
      settings: OpenFcn=open_system([gcb '/Sensor'],'mask')
      mask Help: eval('openHelp(462)')
      mask Display: image(imread('GPS.png'))
  SELF_Sphere_78 : Subsystem  Tag=sensor/SelfPort  Priority=30  LoadFcn=load('PreScanSelfSensorData.mat')  mask(PreScan Source Block: SELF){}
      mask help: The SELF port shows (state) information of the actor itself. The outputs are position in the experiment's axis system and the GPS coordinates, and the object's absolute velocity and compass heading. For more information, please click Help.
      settings: OpenFcn=open_system([gcb '/Sensor'],'mask')
      mask Help: eval('openHelp(462)')
      mask Display: image(imread('GPS.png'))
  SELF_Sphere_79 : Subsystem  Tag=sensor/SelfPort  Priority=30  LoadFcn=load('PreScanSelfSensorData.mat')  mask(PreScan Source Block: SELF){}
      mask help: The SELF port shows (state) information of the actor itself. The outputs are position in the experiment's axis system and the GPS coordinates, and the object's absolute velocity and compass heading. For more information, please click Help.
      settings: OpenFcn=open_system([gcb '/Sensor'],'mask')
      mask Help: eval('openHelp(462)')
      mask Display: image(imread('GPS.png'))
  SELF_Sphere_8 : Subsystem  Tag=sensor/SelfPort  Priority=30  LoadFcn=load('PreScanSelfSensorData.mat')  mask(PreScan Source Block: SELF){}
      mask help: The SELF port shows (state) information of the actor itself. The outputs are position in the experiment's axis system and the GPS coordinates, and the object's absolute velocity and compass heading. For more information, please click Help.
      settings: OpenFcn=open_system([gcb '/Sensor'],'mask')
      mask Help: eval('openHelp(462)')
      mask Display: image(imread('GPS.png'))
  SELF_Sphere_80 : Subsystem  Tag=sensor/SelfPort  Priority=30  LoadFcn=load('PreScanSelfSensorData.mat')  mask(PreScan Source Block: SELF){}
      mask help: The SELF port shows (state) information of the actor itself. The outputs are position in the experiment's axis system and the GPS coordinates, and the object's absolute velocity and compass heading. For more information, please click Help.
      settings: OpenFcn=open_system([gcb '/Sensor'],'mask')
      mask Help: eval('openHelp(462)')
      mask Display: image(imread('GPS.png'))
  SELF_Sphere_81 : Subsystem  Tag=sensor/SelfPort  Priority=30  LoadFcn=load('PreScanSelfSensorData.mat')  mask(PreScan Source Block: SELF){}
      mask help: The SELF port shows (state) information of the actor itself. The outputs are position in the experiment's axis system and the GPS coordinates, and the object's absolute velocity and compass heading. For more information, please click Help.
      settings: OpenFcn=open_system([gcb '/Sensor'],'mask')
      mask Help: eval('openHelp(462)')
      mask Display: image(imread('GPS.png'))
  SELF_Sphere_9 : Subsystem  Tag=sensor/SelfPort  Priority=30  LoadFcn=load('PreScanSelfSensorData.mat')  mask(PreScan Source Block: SELF){}
      mask help: The SELF port shows (state) information of the actor itself. The outputs are position in the experiment's axis system and the GPS coordinates, and the object's absolute velocity and compass heading. For more information, please click Help.
      settings: OpenFcn=open_system([gcb '/Sensor'],'mask')
      mask Help: eval('openHelp(462)')
      mask Display: image(imread('GPS.png'))
  STATE_Cone_1_bus : Subsystem  Tag=actuator/StatePort  Priority=0  LoadFcn=load('PreScanStateActuatorData.mat')  mask(PreScan Sink Block: State){}
      mask help: The Actor State contains a vector signal of size (9x1), containing the following signals: - Position (x,y,z) [m] - Velocity (vx,vy,vz) [m/s] - Angles (Roll, Pitch, Yaw) [rad] The Actor state is defined in the global axis system. The state is superponed on the Initial position defined in the GUI. For more information, please click Help.
      settings: OpenFcn=open_system([gcb '/Actuator'],'mask')
      mask Help: eval('openHelp(222)')
      mask Display: image(imread('State.png'))
  STATE_Cylinder_1_bus : Subsystem  Tag=actuator/StatePort  Priority=0  LoadFcn=load('PreScanStateActuatorData.mat')  mask(PreScan Sink Block: State){}
      mask help: The Actor State contains a vector signal of size (9x1), containing the following signals: - Position (x,y,z) [m] - Velocity (vx,vy,vz) [m/s] - Angles (Roll, Pitch, Yaw) [rad] The Actor state is defined in the global axis system. The state is superponed on the Initial position defined in the GUI. For more information, please click Help.
      settings: OpenFcn=open_system([gcb '/Actuator'],'mask')
      mask Help: eval('openHelp(222)')
      mask Display: image(imread('State.png'))
  STATE_Cylinder_2_bus : Subsystem  Tag=actuator/StatePort  Priority=0  LoadFcn=load('PreScanStateActuatorData.mat')  mask(PreScan Sink Block: State){}
      mask help: The Actor State contains a vector signal of size (9x1), containing the following signals: - Position (x,y,z) [m] - Velocity (vx,vy,vz) [m/s] - Angles (Roll, Pitch, Yaw) [rad] The Actor state is defined in the global axis system. The state is superponed on the Initial position defined in the GUI. For more information, please click Help.
      settings: OpenFcn=open_system([gcb '/Actuator'],'mask')
      mask Help: eval('openHelp(222)')
      mask Display: image(imread('State.png'))
  STATE_Sphere_10_bus : Subsystem  Tag=actuator/StatePort  Priority=0  LoadFcn=load('PreScanStateActuatorData.mat')  mask(PreScan Sink Block: State){}
      mask help: The Actor State contains a vector signal of size (9x1), containing the following signals: - Position (x,y,z) [m] - Velocity (vx,vy,vz) [m/s] - Angles (Roll, Pitch, Yaw) [rad] The Actor state is defined in the global axis system. The state is superponed on the Initial position defined in the GUI. For more information, please click Help.
      settings: OpenFcn=open_system([gcb '/Actuator'],'mask')
      mask Help: eval('openHelp(222)')
      mask Display: image(imread('State.png'))
  STATE_Sphere_11_bus : Subsystem  Tag=actuator/StatePort  Priority=0  LoadFcn=load('PreScanStateActuatorData.mat')  mask(PreScan Sink Block: State){}
      mask help: The Actor State contains a vector signal of size (9x1), containing the following signals: - Position (x,y,z) [m] - Velocity (vx,vy,vz) [m/s] - Angles (Roll, Pitch, Yaw) [rad] The Actor state is defined in the global axis system. The state is superponed on the Initial position defined in the GUI. For more information, please click Help.
      settings: OpenFcn=open_system([gcb '/Actuator'],'mask')
      mask Help: eval('openHelp(222)')
      mask Display: image(imread('State.png'))
  STATE_Sphere_12_bus : Subsystem  Tag=actuator/StatePort  Priority=0  LoadFcn=load('PreScanStateActuatorData.mat')  mask(PreScan Sink Block: State){}
      mask help: The Actor State contains a vector signal of size (9x1), containing the following signals: - Position (x,y,z) [m] - Velocity (vx,vy,vz) [m/s] - Angles (Roll, Pitch, Yaw) [rad] The Actor state is defined in the global axis system. The state is superponed on the Initial position defined in the GUI. For more information, please click Help.
      settings: OpenFcn=open_system([gcb '/Actuator'],'mask')
      mask Help: eval('openHelp(222)')
      mask Display: image(imread('State.png'))
  STATE_Sphere_13_bus : Subsystem  Tag=actuator/StatePort  Priority=0  LoadFcn=load('PreScanStateActuatorData.mat')  mask(PreScan Sink Block: State){}
      mask help: The Actor State contains a vector signal of size (9x1), containing the following signals: - Position (x,y,z) [m] - Velocity (vx,vy,vz) [m/s] - Angles (Roll, Pitch, Yaw) [rad] The Actor state is defined in the global axis system. The state is superponed on the Initial position defined in the GUI. For more information, please click Help.
      settings: OpenFcn=open_system([gcb '/Actuator'],'mask')
      mask Help: eval('openHelp(222)')
      mask Display: image(imread('State.png'))
  STATE_Sphere_14_bus : Subsystem  Tag=actuator/StatePort  Priority=0  LoadFcn=load('PreScanStateActuatorData.mat')  mask(PreScan Sink Block: State){}
      mask help: The Actor State contains a vector signal of size (9x1), containing the following signals: - Position (x,y,z) [m] - Velocity (vx,vy,vz) [m/s] - Angles (Roll, Pitch, Yaw) [rad] The Actor state is defined in the global axis system. The state is superponed on the Initial position defined in the GUI. For more information, please click Help.
      settings: OpenFcn=open_system([gcb '/Actuator'],'mask')
      mask Help: eval('openHelp(222)')
      mask Display: image(imread('State.png'))
  STATE_Sphere_15_bus : Subsystem  Tag=actuator/StatePort  Priority=0  LoadFcn=load('PreScanStateActuatorData.mat')  mask(PreScan Sink Block: State){}
      mask help: The Actor State contains a vector signal of size (9x1), containing the following signals: - Position (x,y,z) [m] - Velocity (vx,vy,vz) [m/s] - Angles (Roll, Pitch, Yaw) [rad] The Actor state is defined in the global axis system. The state is superponed on the Initial position defined in the GUI. For more information, please click Help.
      settings: OpenFcn=open_system([gcb '/Actuator'],'mask')
      mask Help: eval('openHelp(222)')
      mask Display: image(imread('State.png'))
  STATE_Sphere_16_bus : Subsystem  Tag=actuator/StatePort  Priority=0  LoadFcn=load('PreScanStateActuatorData.mat')  mask(PreScan Sink Block: State){}
      mask help: The Actor State contains a vector signal of size (9x1), containing the following signals: - Position (x,y,z) [m] - Velocity (vx,vy,vz) [m/s] - Angles (Roll, Pitch, Yaw) [rad] The Actor state is defined in the global axis system. The state is superponed on the Initial position defined in the GUI. For more information, please click Help.
      settings: OpenFcn=open_system([gcb '/Actuator'],'mask')
      mask Help: eval('openHelp(222)')
      mask Display: image(imread('State.png'))
  STATE_Sphere_17_bus : Subsystem  Tag=actuator/StatePort  Priority=0  LoadFcn=load('PreScanStateActuatorData.mat')  mask(PreScan Sink Block: State){}
      mask help: The Actor State contains a vector signal of size (9x1), containing the following signals: - Position (x,y,z) [m] - Velocity (vx,vy,vz) [m/s] - Angles (Roll, Pitch, Yaw) [rad] The Actor state is defined in the global axis system. The state is superponed on the Initial position defined in the GUI. For more information, please click Help.
      settings: OpenFcn=open_system([gcb '/Actuator'],'mask')
      mask Help: eval('openHelp(222)')
      mask Display: image(imread('State.png'))
  STATE_Sphere_18_bus : Subsystem  Tag=actuator/StatePort  Priority=0  LoadFcn=load('PreScanStateActuatorData.mat')  mask(PreScan Sink Block: State){}
      mask help: The Actor State contains a vector signal of size (9x1), containing the following signals: - Position (x,y,z) [m] - Velocity (vx,vy,vz) [m/s] - Angles (Roll, Pitch, Yaw) [rad] The Actor state is defined in the global axis system. The state is superponed on the Initial position defined in the GUI. For more information, please click Help.
      settings: OpenFcn=open_system([gcb '/Actuator'],'mask')
      mask Help: eval('openHelp(222)')
      mask Display: image(imread('State.png'))
  STATE_Sphere_19_bus : Subsystem  Tag=actuator/StatePort  Priority=0  LoadFcn=load('PreScanStateActuatorData.mat')  mask(PreScan Sink Block: State){}
      mask help: The Actor State contains a vector signal of size (9x1), containing the following signals: - Position (x,y,z) [m] - Velocity (vx,vy,vz) [m/s] - Angles (Roll, Pitch, Yaw) [rad] The Actor state is defined in the global axis system. The state is superponed on the Initial position defined in the GUI. For more information, please click Help.
      settings: OpenFcn=open_system([gcb '/Actuator'],'mask')
      mask Help: eval('openHelp(222)')
      mask Display: image(imread('State.png'))
  STATE_Sphere_1_bus : Subsystem  Tag=actuator/StatePort  Priority=0  LoadFcn=load('PreScanStateActuatorData.mat')  mask(PreScan Sink Block: State){}
      mask help: The Actor State contains a vector signal of size (9x1), containing the following signals: - Position (x,y,z) [m] - Velocity (vx,vy,vz) [m/s] - Angles (Roll, Pitch, Yaw) [rad] The Actor state is defined in the global axis system. The state is superponed on the Initial position defined in the GUI. For more information, please click Help.
      settings: OpenFcn=open_system([gcb '/Actuator'],'mask')
      mask Help: eval('openHelp(222)')
      mask Display: image(imread('State.png'))
  STATE_Sphere_20_bus : Subsystem  Tag=actuator/StatePort  Priority=0  LoadFcn=load('PreScanStateActuatorData.mat')  mask(PreScan Sink Block: State){}
      mask help: The Actor State contains a vector signal of size (9x1), containing the following signals: - Position (x,y,z) [m] - Velocity (vx,vy,vz) [m/s] - Angles (Roll, Pitch, Yaw) [rad] The Actor state is defined in the global axis system. The state is superponed on the Initial position defined in the GUI. For more information, please click Help.
      settings: OpenFcn=open_system([gcb '/Actuator'],'mask')
      mask Help: eval('openHelp(222)')
      mask Display: image(imread('State.png'))
  STATE_Sphere_21_bus : Subsystem  Tag=actuator/StatePort  Priority=0  LoadFcn=load('PreScanStateActuatorData.mat')  mask(PreScan Sink Block: State){}
      mask help: The Actor State contains a vector signal of size (9x1), containing the following signals: - Position (x,y,z) [m] - Velocity (vx,vy,vz) [m/s] - Angles (Roll, Pitch, Yaw) [rad] The Actor state is defined in the global axis system. The state is superponed on the Initial position defined in the GUI. For more information, please click Help.
      settings: OpenFcn=open_system([gcb '/Actuator'],'mask')
      mask Help: eval('openHelp(222)')
      mask Display: image(imread('State.png'))
  STATE_Sphere_22_bus : Subsystem  Tag=actuator/StatePort  Priority=0  LoadFcn=load('PreScanStateActuatorData.mat')  mask(PreScan Sink Block: State){}
      mask help: The Actor State contains a vector signal of size (9x1), containing the following signals: - Position (x,y,z) [m] - Velocity (vx,vy,vz) [m/s] - Angles (Roll, Pitch, Yaw) [rad] The Actor state is defined in the global axis system. The state is superponed on the Initial position defined in the GUI. For more information, please click Help.
      settings: OpenFcn=open_system([gcb '/Actuator'],'mask')
      mask Help: eval('openHelp(222)')
      mask Display: image(imread('State.png'))
  STATE_Sphere_23_bus : Subsystem  Tag=actuator/StatePort  Priority=0  LoadFcn=load('PreScanStateActuatorData.mat')  mask(PreScan Sink Block: State){}
      mask help: The Actor State contains a vector signal of size (9x1), containing the following signals: - Position (x,y,z) [m] - Velocity (vx,vy,vz) [m/s] - Angles (Roll, Pitch, Yaw) [rad] The Actor state is defined in the global axis system. The state is superponed on the Initial position defined in the GUI. For more information, please click Help.
      settings: OpenFcn=open_system([gcb '/Actuator'],'mask')
      mask Help: eval('openHelp(222)')
      mask Display: image(imread('State.png'))
  STATE_Sphere_24_bus : Subsystem  Tag=actuator/StatePort  Priority=0  LoadFcn=load('PreScanStateActuatorData.mat')  mask(PreScan Sink Block: State){}
      mask help: The Actor State contains a vector signal of size (9x1), containing the following signals: - Position (x,y,z) [m] - Velocity (vx,vy,vz) [m/s] - Angles (Roll, Pitch, Yaw) [rad] The Actor state is defined in the global axis system. The state is superponed on the Initial position defined in the GUI. For more information, please click Help.
      settings: OpenFcn=open_system([gcb '/Actuator'],'mask')
      mask Help: eval('openHelp(222)')
      mask Display: image(imread('State.png'))
  STATE_Sphere_25_bus : Subsystem  Tag=actuator/StatePort  Priority=0  LoadFcn=load('PreScanStateActuatorData.mat')  mask(PreScan Sink Block: State){}
      mask help: The Actor State contains a vector signal of size (9x1), containing the following signals: - Position (x,y,z) [m] - Velocity (vx,vy,vz) [m/s] - Angles (Roll, Pitch, Yaw) [rad] The Actor state is defined in the global axis system. The state is superponed on the Initial position defined in the GUI. For more information, please click Help.
      settings: OpenFcn=open_system([gcb '/Actuator'],'mask')
      mask Help: eval('openHelp(222)')
      mask Display: image(imread('State.png'))
  STATE_Sphere_26_bus : Subsystem  Tag=actuator/StatePort  Priority=0  LoadFcn=load('PreScanStateActuatorData.mat')  mask(PreScan Sink Block: State){}
      mask help: The Actor State contains a vector signal of size (9x1), containing the following signals: - Position (x,y,z) [m] - Velocity (vx,vy,vz) [m/s] - Angles (Roll, Pitch, Yaw) [rad] The Actor state is defined in the global axis system. The state is superponed on the Initial position defined in the GUI. For more information, please click Help.
      settings: OpenFcn=open_system([gcb '/Actuator'],'mask')
      mask Help: eval('openHelp(222)')
      mask Display: image(imread('State.png'))
  STATE_Sphere_27_bus : Subsystem  Tag=actuator/StatePort  Priority=0  LoadFcn=load('PreScanStateActuatorData.mat')  mask(PreScan Sink Block: State){}
      mask help: The Actor State contains a vector signal of size (9x1), containing the following signals: - Position (x,y,z) [m] - Velocity (vx,vy,vz) [m/s] - Angles (Roll, Pitch, Yaw) [rad] The Actor state is defined in the global axis system. The state is superponed on the Initial position defined in the GUI. For more information, please click Help.
      settings: OpenFcn=open_system([gcb '/Actuator'],'mask')
      mask Help: eval('openHelp(222)')
      mask Display: image(imread('State.png'))
  STATE_Sphere_28_bus : Subsystem  Tag=actuator/StatePort  Priority=0  LoadFcn=load('PreScanStateActuatorData.mat')  mask(PreScan Sink Block: State){}
      mask help: The Actor State contains a vector signal of size (9x1), containing the following signals: - Position (x,y,z) [m] - Velocity (vx,vy,vz) [m/s] - Angles (Roll, Pitch, Yaw) [rad] The Actor state is defined in the global axis system. The state is superponed on the Initial position defined in the GUI. For more information, please click Help.
      settings: OpenFcn=open_system([gcb '/Actuator'],'mask')
      mask Help: eval('openHelp(222)')
      mask Display: image(imread('State.png'))
  STATE_Sphere_29_bus : Subsystem  Tag=actuator/StatePort  Priority=0  LoadFcn=load('PreScanStateActuatorData.mat')  mask(PreScan Sink Block: State){}
      mask help: The Actor State contains a vector signal of size (9x1), containing the following signals: - Position (x,y,z) [m] - Velocity (vx,vy,vz) [m/s] - Angles (Roll, Pitch, Yaw) [rad] The Actor state is defined in the global axis system. The state is superponed on the Initial position defined in the GUI. For more information, please click Help.
      settings: OpenFcn=open_system([gcb '/Actuator'],'mask')
      mask Help: eval('openHelp(222)')
      mask Display: image(imread('State.png'))
  STATE_Sphere_2_bus : Subsystem  Tag=actuator/StatePort  Priority=0  LoadFcn=load('PreScanStateActuatorData.mat')  mask(PreScan Sink Block: State){}
      mask help: The Actor State contains a vector signal of size (9x1), containing the following signals: - Position (x,y,z) [m] - Velocity (vx,vy,vz) [m/s] - Angles (Roll, Pitch, Yaw) [rad] The Actor state is defined in the global axis system. The state is superponed on the Initial position defined in the GUI. For more information, please click Help.
      settings: OpenFcn=open_system([gcb '/Actuator'],'mask')
      mask Help: eval('openHelp(222)')
      mask Display: image(imread('State.png'))
  STATE_Sphere_30_bus : Subsystem  Tag=actuator/StatePort  Priority=0  LoadFcn=load('PreScanStateActuatorData.mat')  mask(PreScan Sink Block: State){}
      mask help: The Actor State contains a vector signal of size (9x1), containing the following signals: - Position (x,y,z) [m] - Velocity (vx,vy,vz) [m/s] - Angles (Roll, Pitch, Yaw) [rad] The Actor state is defined in the global axis system. The state is superponed on the Initial position defined in the GUI. For more information, please click Help.
      settings: OpenFcn=open_system([gcb '/Actuator'],'mask')
      mask Help: eval('openHelp(222)')
      mask Display: image(imread('State.png'))
  STATE_Sphere_31_bus : Subsystem  Tag=actuator/StatePort  Priority=0  LoadFcn=load('PreScanStateActuatorData.mat')  mask(PreScan Sink Block: State){}
      mask help: The Actor State contains a vector signal of size (9x1), containing the following signals: - Position (x,y,z) [m] - Velocity (vx,vy,vz) [m/s] - Angles (Roll, Pitch, Yaw) [rad] The Actor state is defined in the global axis system. The state is superponed on the Initial position defined in the GUI. For more information, please click Help.
      settings: OpenFcn=open_system([gcb '/Actuator'],'mask')
      mask Help: eval('openHelp(222)')
      mask Display: image(imread('State.png'))
  STATE_Sphere_32_bus : Subsystem  Tag=actuator/StatePort  Priority=0  LoadFcn=load('PreScanStateActuatorData.mat')  mask(PreScan Sink Block: State){}
      mask help: The Actor State contains a vector signal of size (9x1), containing the following signals: - Position (x,y,z) [m] - Velocity (vx,vy,vz) [m/s] - Angles (Roll, Pitch, Yaw) [rad] The Actor state is defined in the global axis system. The state is superponed on the Initial position defined in the GUI. For more information, please click Help.
      settings: OpenFcn=open_system([gcb '/Actuator'],'mask')
      mask Help: eval('openHelp(222)')
      mask Display: image(imread('State.png'))
  STATE_Sphere_33_bus : Subsystem  Tag=actuator/StatePort  Priority=0  LoadFcn=load('PreScanStateActuatorData.mat')  mask(PreScan Sink Block: State){}
      mask help: The Actor State contains a vector signal of size (9x1), containing the following signals: - Position (x,y,z) [m] - Velocity (vx,vy,vz) [m/s] - Angles (Roll, Pitch, Yaw) [rad] The Actor state is defined in the global axis system. The state is superponed on the Initial position defined in the GUI. For more information, please click Help.
      settings: OpenFcn=open_system([gcb '/Actuator'],'mask')
      mask Help: eval('openHelp(222)')
      mask Display: image(imread('State.png'))
  STATE_Sphere_34_bus : Subsystem  Tag=actuator/StatePort  Priority=0  LoadFcn=load('PreScanStateActuatorData.mat')  mask(PreScan Sink Block: State){}
      mask help: The Actor State contains a vector signal of size (9x1), containing the following signals: - Position (x,y,z) [m] - Velocity (vx,vy,vz) [m/s] - Angles (Roll, Pitch, Yaw) [rad] The Actor state is defined in the global axis system. The state is superponed on the Initial position defined in the GUI. For more information, please click Help.
      settings: OpenFcn=open_system([gcb '/Actuator'],'mask')
      mask Help: eval('openHelp(222)')
      mask Display: image(imread('State.png'))
  STATE_Sphere_35_bus : Subsystem  Tag=actuator/StatePort  Priority=0  LoadFcn=load('PreScanStateActuatorData.mat')  mask(PreScan Sink Block: State){}
      mask help: The Actor State contains a vector signal of size (9x1), containing the following signals: - Position (x,y,z) [m] - Velocity (vx,vy,vz) [m/s] - Angles (Roll, Pitch, Yaw) [rad] The Actor state is defined in the global axis system. The state is superponed on the Initial position defined in the GUI. For more information, please click Help.
      settings: OpenFcn=open_system([gcb '/Actuator'],'mask')
      mask Help: eval('openHelp(222)')
      mask Display: image(imread('State.png'))
  STATE_Sphere_36_bus : Subsystem  Tag=actuator/StatePort  Priority=0  LoadFcn=load('PreScanStateActuatorData.mat')  mask(PreScan Sink Block: State){}
      mask help: The Actor State contains a vector signal of size (9x1), containing the following signals: - Position (x,y,z) [m] - Velocity (vx,vy,vz) [m/s] - Angles (Roll, Pitch, Yaw) [rad] The Actor state is defined in the global axis system. The state is superponed on the Initial position defined in the GUI. For more information, please click Help.
      settings: OpenFcn=open_system([gcb '/Actuator'],'mask')
      mask Help: eval('openHelp(222)')
      mask Display: image(imread('State.png'))
  STATE_Sphere_37_bus : Subsystem  Tag=actuator/StatePort  Priority=0  LoadFcn=load('PreScanStateActuatorData.mat')  mask(PreScan Sink Block: State){}
      mask help: The Actor State contains a vector signal of size (9x1), containing the following signals: - Position (x,y,z) [m] - Velocity (vx,vy,vz) [m/s] - Angles (Roll, Pitch, Yaw) [rad] The Actor state is defined in the global axis system. The state is superponed on the Initial position defined in the GUI. For more information, please click Help.
      settings: OpenFcn=open_system([gcb '/Actuator'],'mask')
      mask Help: eval('openHelp(222)')
      mask Display: image(imread('State.png'))
  STATE_Sphere_38_bus : Subsystem  Tag=actuator/StatePort  Priority=0  LoadFcn=load('PreScanStateActuatorData.mat')  mask(PreScan Sink Block: State){}
      mask help: The Actor State contains a vector signal of size (9x1), containing the following signals: - Position (x,y,z) [m] - Velocity (vx,vy,vz) [m/s] - Angles (Roll, Pitch, Yaw) [rad] The Actor state is defined in the global axis system. The state is superponed on the Initial position defined in the GUI. For more information, please click Help.
      settings: OpenFcn=open_system([gcb '/Actuator'],'mask')
      mask Help: eval('openHelp(222)')
      mask Display: image(imread('State.png'))
  STATE_Sphere_39_bus : Subsystem  Tag=actuator/StatePort  Priority=0  LoadFcn=load('PreScanStateActuatorData.mat')  mask(PreScan Sink Block: State){}
      mask help: The Actor State contains a vector signal of size (9x1), containing the following signals: - Position (x,y,z) [m] - Velocity (vx,vy,vz) [m/s] - Angles (Roll, Pitch, Yaw) [rad] The Actor state is defined in the global axis system. The state is superponed on the Initial position defined in the GUI. For more information, please click Help.
      settings: OpenFcn=open_system([gcb '/Actuator'],'mask')
      mask Help: eval('openHelp(222)')
      mask Display: image(imread('State.png'))
  STATE_Sphere_3_bus : Subsystem  Tag=actuator/StatePort  Priority=0  LoadFcn=load('PreScanStateActuatorData.mat')  mask(PreScan Sink Block: State){}
      mask help: The Actor State contains a vector signal of size (9x1), containing the following signals: - Position (x,y,z) [m] - Velocity (vx,vy,vz) [m/s] - Angles (Roll, Pitch, Yaw) [rad] The Actor state is defined in the global axis system. The state is superponed on the Initial position defined in the GUI. For more information, please click Help.
      settings: OpenFcn=open_system([gcb '/Actuator'],'mask')
      mask Help: eval('openHelp(222)')
      mask Display: image(imread('State.png'))
  STATE_Sphere_40_bus : Subsystem  Tag=actuator/StatePort  Priority=0  LoadFcn=load('PreScanStateActuatorData.mat')  mask(PreScan Sink Block: State){}
      mask help: The Actor State contains a vector signal of size (9x1), containing the following signals: - Position (x,y,z) [m] - Velocity (vx,vy,vz) [m/s] - Angles (Roll, Pitch, Yaw) [rad] The Actor state is defined in the global axis system. The state is superponed on the Initial position defined in the GUI. For more information, please click Help.
      settings: OpenFcn=open_system([gcb '/Actuator'],'mask')
      mask Help: eval('openHelp(222)')
      mask Display: image(imread('State.png'))
  STATE_Sphere_41_bus : Subsystem  Tag=actuator/StatePort  Priority=0  LoadFcn=load('PreScanStateActuatorData.mat')  mask(PreScan Sink Block: State){}
      mask help: The Actor State contains a vector signal of size (9x1), containing the following signals: - Position (x,y,z) [m] - Velocity (vx,vy,vz) [m/s] - Angles (Roll, Pitch, Yaw) [rad] The Actor state is defined in the global axis system. The state is superponed on the Initial position defined in the GUI. For more information, please click Help.
      settings: OpenFcn=open_system([gcb '/Actuator'],'mask')
      mask Help: eval('openHelp(222)')
      mask Display: image(imread('State.png'))
  STATE_Sphere_42_bus : Subsystem  Tag=actuator/StatePort  Priority=0  LoadFcn=load('PreScanStateActuatorData.mat')  mask(PreScan Sink Block: State){}
      mask help: The Actor State contains a vector signal of size (9x1), containing the following signals: - Position (x,y,z) [m] - Velocity (vx,vy,vz) [m/s] - Angles (Roll, Pitch, Yaw) [rad] The Actor state is defined in the global axis system. The state is superponed on the Initial position defined in the GUI. For more information, please click Help.
      settings: OpenFcn=open_system([gcb '/Actuator'],'mask')
      mask Help: eval('openHelp(222)')
      mask Display: image(imread('State.png'))
  STATE_Sphere_43_bus : Subsystem  Tag=actuator/StatePort  Priority=0  LoadFcn=load('PreScanStateActuatorData.mat')  mask(PreScan Sink Block: State){}
      mask help: The Actor State contains a vector signal of size (9x1), containing the following signals: - Position (x,y,z) [m] - Velocity (vx,vy,vz) [m/s] - Angles (Roll, Pitch, Yaw) [rad] The Actor state is defined in the global axis system. The state is superponed on the Initial position defined in the GUI. For more information, please click Help.
      settings: OpenFcn=open_system([gcb '/Actuator'],'mask')
      mask Help: eval('openHelp(222)')
      mask Display: image(imread('State.png'))
  STATE_Sphere_44_bus : Subsystem  Tag=actuator/StatePort  Priority=0  LoadFcn=load('PreScanStateActuatorData.mat')  mask(PreScan Sink Block: State){}
      mask help: The Actor State contains a vector signal of size (9x1), containing the following signals: - Position (x,y,z) [m] - Velocity (vx,vy,vz) [m/s] - Angles (Roll, Pitch, Yaw) [rad] The Actor state is defined in the global axis system. The state is superponed on the Initial position defined in the GUI. For more information, please click Help.
      settings: OpenFcn=open_system([gcb '/Actuator'],'mask')
      mask Help: eval('openHelp(222)')
      mask Display: image(imread('State.png'))
  STATE_Sphere_45_bus : Subsystem  Tag=actuator/StatePort  Priority=0  LoadFcn=load('PreScanStateActuatorData.mat')  mask(PreScan Sink Block: State){}
      mask help: The Actor State contains a vector signal of size (9x1), containing the following signals: - Position (x,y,z) [m] - Velocity (vx,vy,vz) [m/s] - Angles (Roll, Pitch, Yaw) [rad] The Actor state is defined in the global axis system. The state is superponed on the Initial position defined in the GUI. For more information, please click Help.
      settings: OpenFcn=open_system([gcb '/Actuator'],'mask')
      mask Help: eval('openHelp(222)')
      mask Display: image(imread('State.png'))
  STATE_Sphere_46_bus : Subsystem  Tag=actuator/StatePort  Priority=0  LoadFcn=load('PreScanStateActuatorData.mat')  mask(PreScan Sink Block: State){}
      mask help: The Actor State contains a vector signal of size (9x1), containing the following signals: - Position (x,y,z) [m] - Velocity (vx,vy,vz) [m/s] - Angles (Roll, Pitch, Yaw) [rad] The Actor state is defined in the global axis system. The state is superponed on the Initial position defined in the GUI. For more information, please click Help.
      settings: OpenFcn=open_system([gcb '/Actuator'],'mask')
      mask Help: eval('openHelp(222)')
      mask Display: image(imread('State.png'))
  STATE_Sphere_47_bus : Subsystem  Tag=actuator/StatePort  Priority=0  LoadFcn=load('PreScanStateActuatorData.mat')  mask(PreScan Sink Block: State){}
      mask help: The Actor State contains a vector signal of size (9x1), containing the following signals: - Position (x,y,z) [m] - Velocity (vx,vy,vz) [m/s] - Angles (Roll, Pitch, Yaw) [rad] The Actor state is defined in the global axis system. The state is superponed on the Initial position defined in the GUI. For more information, please click Help.
      settings: OpenFcn=open_system([gcb '/Actuator'],'mask')
      mask Help: eval('openHelp(222)')
      mask Display: image(imread('State.png'))
  STATE_Sphere_48_bus : Subsystem  Tag=actuator/StatePort  Priority=0  LoadFcn=load('PreScanStateActuatorData.mat')  mask(PreScan Sink Block: State){}
      mask help: The Actor State contains a vector signal of size (9x1), containing the following signals: - Position (x,y,z) [m] - Velocity (vx,vy,vz) [m/s] - Angles (Roll, Pitch, Yaw) [rad] The Actor state is defined in the global axis system. The state is superponed on the Initial position defined in the GUI. For more information, please click Help.
      settings: OpenFcn=open_system([gcb '/Actuator'],'mask')
      mask Help: eval('openHelp(222)')
      mask Display: image(imread('State.png'))
  STATE_Sphere_49_bus : Subsystem  Tag=actuator/StatePort  Priority=0  LoadFcn=load('PreScanStateActuatorData.mat')  mask(PreScan Sink Block: State){}
      mask help: The Actor State contains a vector signal of size (9x1), containing the following signals: - Position (x,y,z) [m] - Velocity (vx,vy,vz) [m/s] - Angles (Roll, Pitch, Yaw) [rad] The Actor state is defined in the global axis system. The state is superponed on the Initial position defined in the GUI. For more information, please click Help.
      settings: OpenFcn=open_system([gcb '/Actuator'],'mask')
      mask Help: eval('openHelp(222)')
      mask Display: image(imread('State.png'))
  STATE_Sphere_4_bus : Subsystem  Tag=actuator/StatePort  Priority=0  LoadFcn=load('PreScanStateActuatorData.mat')  mask(PreScan Sink Block: State){}
      mask help: The Actor State contains a vector signal of size (9x1), containing the following signals: - Position (x,y,z) [m] - Velocity (vx,vy,vz) [m/s] - Angles (Roll, Pitch, Yaw) [rad] The Actor state is defined in the global axis system. The state is superponed on the Initial position defined in the GUI. For more information, please click Help.
      settings: OpenFcn=open_system([gcb '/Actuator'],'mask')
      mask Help: eval('openHelp(222)')
      mask Display: image(imread('State.png'))
  STATE_Sphere_50_bus : Subsystem  Tag=actuator/StatePort  Priority=0  LoadFcn=load('PreScanStateActuatorData.mat')  mask(PreScan Sink Block: State){}
      mask help: The Actor State contains a vector signal of size (9x1), containing the following signals: - Position (x,y,z) [m] - Velocity (vx,vy,vz) [m/s] - Angles (Roll, Pitch, Yaw) [rad] The Actor state is defined in the global axis system. The state is superponed on the Initial position defined in the GUI. For more information, please click Help.
      settings: OpenFcn=open_system([gcb '/Actuator'],'mask')
      mask Help: eval('openHelp(222)')
      mask Display: image(imread('State.png'))
  STATE_Sphere_51_bus : Subsystem  Tag=actuator/StatePort  Priority=0  LoadFcn=load('PreScanStateActuatorData.mat')  mask(PreScan Sink Block: State){}
      mask help: The Actor State contains a vector signal of size (9x1), containing the following signals: - Position (x,y,z) [m] - Velocity (vx,vy,vz) [m/s] - Angles (Roll, Pitch, Yaw) [rad] The Actor state is defined in the global axis system. The state is superponed on the Initial position defined in the GUI. For more information, please click Help.
      settings: OpenFcn=open_system([gcb '/Actuator'],'mask')
      mask Help: eval('openHelp(222)')
      mask Display: image(imread('State.png'))
  STATE_Sphere_52_bus : Subsystem  Tag=actuator/StatePort  Priority=0  LoadFcn=load('PreScanStateActuatorData.mat')  mask(PreScan Sink Block: State){}
      mask help: The Actor State contains a vector signal of size (9x1), containing the following signals: - Position (x,y,z) [m] - Velocity (vx,vy,vz) [m/s] - Angles (Roll, Pitch, Yaw) [rad] The Actor state is defined in the global axis system. The state is superponed on the Initial position defined in the GUI. For more information, please click Help.
      settings: OpenFcn=open_system([gcb '/Actuator'],'mask')
      mask Help: eval('openHelp(222)')
      mask Display: image(imread('State.png'))
  STATE_Sphere_53_bus : Subsystem  Tag=actuator/StatePort  Priority=0  LoadFcn=load('PreScanStateActuatorData.mat')  mask(PreScan Sink Block: State){}
      mask help: The Actor State contains a vector signal of size (9x1), containing the following signals: - Position (x,y,z) [m] - Velocity (vx,vy,vz) [m/s] - Angles (Roll, Pitch, Yaw) [rad] The Actor state is defined in the global axis system. The state is superponed on the Initial position defined in the GUI. For more information, please click Help.
      settings: OpenFcn=open_system([gcb '/Actuator'],'mask')
      mask Help: eval('openHelp(222)')
      mask Display: image(imread('State.png'))
  STATE_Sphere_54_bus : Subsystem  Tag=actuator/StatePort  Priority=0  LoadFcn=load('PreScanStateActuatorData.mat')  mask(PreScan Sink Block: State){}
      mask help: The Actor State contains a vector signal of size (9x1), containing the following signals: - Position (x,y,z) [m] - Velocity (vx,vy,vz) [m/s] - Angles (Roll, Pitch, Yaw) [rad] The Actor state is defined in the global axis system. The state is superponed on the Initial position defined in the GUI. For more information, please click Help.
      settings: OpenFcn=open_system([gcb '/Actuator'],'mask')
      mask Help: eval('openHelp(222)')
      mask Display: image(imread('State.png'))
  STATE_Sphere_55_bus : Subsystem  Tag=actuator/StatePort  Priority=0  LoadFcn=load('PreScanStateActuatorData.mat')  mask(PreScan Sink Block: State){}
      mask help: The Actor State contains a vector signal of size (9x1), containing the following signals: - Position (x,y,z) [m] - Velocity (vx,vy,vz) [m/s] - Angles (Roll, Pitch, Yaw) [rad] The Actor state is defined in the global axis system. The state is superponed on the Initial position defined in the GUI. For more information, please click Help.
      settings: OpenFcn=open_system([gcb '/Actuator'],'mask')
      mask Help: eval('openHelp(222)')
      mask Display: image(imread('State.png'))
  STATE_Sphere_56_bus : Subsystem  Tag=actuator/StatePort  Priority=0  LoadFcn=load('PreScanStateActuatorData.mat')  mask(PreScan Sink Block: State){}
      mask help: The Actor State contains a vector signal of size (9x1), containing the following signals: - Position (x,y,z) [m] - Velocity (vx,vy,vz) [m/s] - Angles (Roll, Pitch, Yaw) [rad] The Actor state is defined in the global axis system. The state is superponed on the Initial position defined in the GUI. For more information, please click Help.
      settings: OpenFcn=open_system([gcb '/Actuator'],'mask')
      mask Help: eval('openHelp(222)')
      mask Display: image(imread('State.png'))
  STATE_Sphere_57_bus : Subsystem  Tag=actuator/StatePort  Priority=0  LoadFcn=load('PreScanStateActuatorData.mat')  mask(PreScan Sink Block: State){}
      mask help: The Actor State contains a vector signal of size (9x1), containing the following signals: - Position (x,y,z) [m] - Velocity (vx,vy,vz) [m/s] - Angles (Roll, Pitch, Yaw) [rad] The Actor state is defined in the global axis system. The state is superponed on the Initial position defined in the GUI. For more information, please click Help.
      settings: OpenFcn=open_system([gcb '/Actuator'],'mask')
      mask Help: eval('openHelp(222)')
      mask Display: image(imread('State.png'))
  STATE_Sphere_58_bus : Subsystem  Tag=actuator/StatePort  Priority=0  LoadFcn=load('PreScanStateActuatorData.mat')  mask(PreScan Sink Block: State){}
      mask help: The Actor State contains a vector signal of size (9x1), containing the following signals: - Position (x,y,z) [m] - Velocity (vx,vy,vz) [m/s] - Angles (Roll, Pitch, Yaw) [rad] The Actor state is defined in the global axis system. The state is superponed on the Initial position defined in the GUI. For more information, please click Help.
      settings: OpenFcn=open_system([gcb '/Actuator'],'mask')
      mask Help: eval('openHelp(222)')
      mask Display: image(imread('State.png'))
  STATE_Sphere_59_bus : Subsystem  Tag=actuator/StatePort  Priority=0  LoadFcn=load('PreScanStateActuatorData.mat')  mask(PreScan Sink Block: State){}
      mask help: The Actor State contains a vector signal of size (9x1), containing the following signals: - Position (x,y,z) [m] - Velocity (vx,vy,vz) [m/s] - Angles (Roll, Pitch, Yaw) [rad] The Actor state is defined in the global axis system. The state is superponed on the Initial position defined in the GUI. For more information, please click Help.
      settings: OpenFcn=open_system([gcb '/Actuator'],'mask')
      mask Help: eval('openHelp(222)')
      mask Display: image(imread('State.png'))
  STATE_Sphere_5_bus : Subsystem  Tag=actuator/StatePort  Priority=0  LoadFcn=load('PreScanStateActuatorData.mat')  mask(PreScan Sink Block: State){}
      mask help: The Actor State contains a vector signal of size (9x1), containing the following signals: - Position (x,y,z) [m] - Velocity (vx,vy,vz) [m/s] - Angles (Roll, Pitch, Yaw) [rad] The Actor state is defined in the global axis system. The state is superponed on the Initial position defined in the GUI. For more information, please click Help.
      settings: OpenFcn=open_system([gcb '/Actuator'],'mask')
      mask Help: eval('openHelp(222)')
      mask Display: image(imread('State.png'))
  STATE_Sphere_60_bus : Subsystem  Tag=actuator/StatePort  Priority=0  LoadFcn=load('PreScanStateActuatorData.mat')  mask(PreScan Sink Block: State){}
      mask help: The Actor State contains a vector signal of size (9x1), containing the following signals: - Position (x,y,z) [m] - Velocity (vx,vy,vz) [m/s] - Angles (Roll, Pitch, Yaw) [rad] The Actor state is defined in the global axis system. The state is superponed on the Initial position defined in the GUI. For more information, please click Help.
      settings: OpenFcn=open_system([gcb '/Actuator'],'mask')
      mask Help: eval('openHelp(222)')
      mask Display: image(imread('State.png'))
  STATE_Sphere_61_bus : Subsystem  Tag=actuator/StatePort  Priority=0  LoadFcn=load('PreScanStateActuatorData.mat')  mask(PreScan Sink Block: State){}
      mask help: The Actor State contains a vector signal of size (9x1), containing the following signals: - Position (x,y,z) [m] - Velocity (vx,vy,vz) [m/s] - Angles (Roll, Pitch, Yaw) [rad] The Actor state is defined in the global axis system. The state is superponed on the Initial position defined in the GUI. For more information, please click Help.
      settings: OpenFcn=open_system([gcb '/Actuator'],'mask')
      mask Help: eval('openHelp(222)')
      mask Display: image(imread('State.png'))
  STATE_Sphere_62_bus : Subsystem  Tag=actuator/StatePort  Priority=0  LoadFcn=load('PreScanStateActuatorData.mat')  mask(PreScan Sink Block: State){}
      mask help: The Actor State contains a vector signal of size (9x1), containing the following signals: - Position (x,y,z) [m] - Velocity (vx,vy,vz) [m/s] - Angles (Roll, Pitch, Yaw) [rad] The Actor state is defined in the global axis system. The state is superponed on the Initial position defined in the GUI. For more information, please click Help.
      settings: OpenFcn=open_system([gcb '/Actuator'],'mask')
      mask Help: eval('openHelp(222)')
      mask Display: image(imread('State.png'))
  STATE_Sphere_63_bus : Subsystem  Tag=actuator/StatePort  Priority=0  LoadFcn=load('PreScanStateActuatorData.mat')  mask(PreScan Sink Block: State){}
      mask help: The Actor State contains a vector signal of size (9x1), containing the following signals: - Position (x,y,z) [m] - Velocity (vx,vy,vz) [m/s] - Angles (Roll, Pitch, Yaw) [rad] The Actor state is defined in the global axis system. The state is superponed on the Initial position defined in the GUI. For more information, please click Help.
      settings: OpenFcn=open_system([gcb '/Actuator'],'mask')
      mask Help: eval('openHelp(222)')
      mask Display: image(imread('State.png'))
  STATE_Sphere_64_bus : Subsystem  Tag=actuator/StatePort  Priority=0  LoadFcn=load('PreScanStateActuatorData.mat')  mask(PreScan Sink Block: State){}
      mask help: The Actor State contains a vector signal of size (9x1), containing the following signals: - Position (x,y,z) [m] - Velocity (vx,vy,vz) [m/s] - Angles (Roll, Pitch, Yaw) [rad] The Actor state is defined in the global axis system. The state is superponed on the Initial position defined in the GUI. For more information, please click Help.
      settings: OpenFcn=open_system([gcb '/Actuator'],'mask')
      mask Help: eval('openHelp(222)')
      mask Display: image(imread('State.png'))
  STATE_Sphere_65_bus : Subsystem  Tag=actuator/StatePort  Priority=0  LoadFcn=load('PreScanStateActuatorData.mat')  mask(PreScan Sink Block: State){}
      mask help: The Actor State contains a vector signal of size (9x1), containing the following signals: - Position (x,y,z) [m] - Velocity (vx,vy,vz) [m/s] - Angles (Roll, Pitch, Yaw) [rad] The Actor state is defined in the global axis system. The state is superponed on the Initial position defined in the GUI. For more information, please click Help.
      settings: OpenFcn=open_system([gcb '/Actuator'],'mask')
      mask Help: eval('openHelp(222)')
      mask Display: image(imread('State.png'))
  STATE_Sphere_66_bus : Subsystem  Tag=actuator/StatePort  Priority=0  LoadFcn=load('PreScanStateActuatorData.mat')  mask(PreScan Sink Block: State){}
      mask help: The Actor State contains a vector signal of size (9x1), containing the following signals: - Position (x,y,z) [m] - Velocity (vx,vy,vz) [m/s] - Angles (Roll, Pitch, Yaw) [rad] The Actor state is defined in the global axis system. The state is superponed on the Initial position defined in the GUI. For more information, please click Help.
      settings: OpenFcn=open_system([gcb '/Actuator'],'mask')
      mask Help: eval('openHelp(222)')
      mask Display: image(imread('State.png'))
  STATE_Sphere_67_bus : Subsystem  Tag=actuator/StatePort  Priority=0  LoadFcn=load('PreScanStateActuatorData.mat')  mask(PreScan Sink Block: State){}
      mask help: The Actor State contains a vector signal of size (9x1), containing the following signals: - Position (x,y,z) [m] - Velocity (vx,vy,vz) [m/s] - Angles (Roll, Pitch, Yaw) [rad] The Actor state is defined in the global axis system. The state is superponed on the Initial position defined in the GUI. For more information, please click Help.
      settings: OpenFcn=open_system([gcb '/Actuator'],'mask')
      mask Help: eval('openHelp(222)')
      mask Display: image(imread('State.png'))
  STATE_Sphere_68_bus : Subsystem  Tag=actuator/StatePort  Priority=0  LoadFcn=load('PreScanStateActuatorData.mat')  mask(PreScan Sink Block: State){}
      mask help: The Actor State contains a vector signal of size (9x1), containing the following signals: - Position (x,y,z) [m] - Velocity (vx,vy,vz) [m/s] - Angles (Roll, Pitch, Yaw) [rad] The Actor state is defined in the global axis system. The state is superponed on the Initial position defined in the GUI. For more information, please click Help.
      settings: OpenFcn=open_system([gcb '/Actuator'],'mask')
      mask Help: eval('openHelp(222)')
      mask Display: image(imread('State.png'))
  STATE_Sphere_69_bus : Subsystem  Tag=actuator/StatePort  Priority=0  LoadFcn=load('PreScanStateActuatorData.mat')  mask(PreScan Sink Block: State){}
      mask help: The Actor State contains a vector signal of size (9x1), containing the following signals: - Position (x,y,z) [m] - Velocity (vx,vy,vz) [m/s] - Angles (Roll, Pitch, Yaw) [rad] The Actor state is defined in the global axis system. The state is superponed on the Initial position defined in the GUI. For more information, please click Help.
      settings: OpenFcn=open_system([gcb '/Actuator'],'mask')
      mask Help: eval('openHelp(222)')
      mask Display: image(imread('State.png'))
  STATE_Sphere_6_bus : Subsystem  Tag=actuator/StatePort  Priority=0  LoadFcn=load('PreScanStateActuatorData.mat')  mask(PreScan Sink Block: State){}
      mask help: The Actor State contains a vector signal of size (9x1), containing the following signals: - Position (x,y,z) [m] - Velocity (vx,vy,vz) [m/s] - Angles (Roll, Pitch, Yaw) [rad] The Actor state is defined in the global axis system. The state is superponed on the Initial position defined in the GUI. For more information, please click Help.
      settings: OpenFcn=open_system([gcb '/Actuator'],'mask')
      mask Help: eval('openHelp(222)')
      mask Display: image(imread('State.png'))
  STATE_Sphere_70_bus : Subsystem  Tag=actuator/StatePort  Priority=0  LoadFcn=load('PreScanStateActuatorData.mat')  mask(PreScan Sink Block: State){}
      mask help: The Actor State contains a vector signal of size (9x1), containing the following signals: - Position (x,y,z) [m] - Velocity (vx,vy,vz) [m/s] - Angles (Roll, Pitch, Yaw) [rad] The Actor state is defined in the global axis system. The state is superponed on the Initial position defined in the GUI. For more information, please click Help.
      settings: OpenFcn=open_system([gcb '/Actuator'],'mask')
      mask Help: eval('openHelp(222)')
      mask Display: image(imread('State.png'))
  STATE_Sphere_71_bus : Subsystem  Tag=actuator/StatePort  Priority=0  LoadFcn=load('PreScanStateActuatorData.mat')  mask(PreScan Sink Block: State){}
      mask help: The Actor State contains a vector signal of size (9x1), containing the following signals: - Position (x,y,z) [m] - Velocity (vx,vy,vz) [m/s] - Angles (Roll, Pitch, Yaw) [rad] The Actor state is defined in the global axis system. The state is superponed on the Initial position defined in the GUI. For more information, please click Help.
      settings: OpenFcn=open_system([gcb '/Actuator'],'mask')
      mask Help: eval('openHelp(222)')
      mask Display: image(imread('State.png'))
  STATE_Sphere_72_bus : Subsystem  Tag=actuator/StatePort  Priority=0  LoadFcn=load('PreScanStateActuatorData.mat')  mask(PreScan Sink Block: State){}
      mask help: The Actor State contains a vector signal of size (9x1), containing the following signals: - Position (x,y,z) [m] - Velocity (vx,vy,vz) [m/s] - Angles (Roll, Pitch, Yaw) [rad] The Actor state is defined in the global axis system. The state is superponed on the Initial position defined in the GUI. For more information, please click Help.
      settings: OpenFcn=open_system([gcb '/Actuator'],'mask')
      mask Help: eval('openHelp(222)')
      mask Display: image(imread('State.png'))
  STATE_Sphere_73_bus : Subsystem  Tag=actuator/StatePort  Priority=0  LoadFcn=load('PreScanStateActuatorData.mat')  mask(PreScan Sink Block: State){}
      mask help: The Actor State contains a vector signal of size (9x1), containing the following signals: - Position (x,y,z) [m] - Velocity (vx,vy,vz) [m/s] - Angles (Roll, Pitch, Yaw) [rad] The Actor state is defined in the global axis system. The state is superponed on the Initial position defined in the GUI. For more information, please click Help.
      settings: OpenFcn=open_system([gcb '/Actuator'],'mask')
      mask Help: eval('openHelp(222)')
      mask Display: image(imread('State.png'))
  STATE_Sphere_74_bus : Subsystem  Tag=actuator/StatePort  Priority=0  LoadFcn=load('PreScanStateActuatorData.mat')  mask(PreScan Sink Block: State){}
      mask help: The Actor State contains a vector signal of size (9x1), containing the following signals: - Position (x,y,z) [m] - Velocity (vx,vy,vz) [m/s] - Angles (Roll, Pitch, Yaw) [rad] The Actor state is defined in the global axis system. The state is superponed on the Initial position defined in the GUI. For more information, please click Help.
      settings: OpenFcn=open_system([gcb '/Actuator'],'mask')
      mask Help: eval('openHelp(222)')
      mask Display: image(imread('State.png'))
  STATE_Sphere_75_bus : Subsystem  Tag=actuator/StatePort  Priority=0  LoadFcn=load('PreScanStateActuatorData.mat')  mask(PreScan Sink Block: State){}
      mask help: The Actor State contains a vector signal of size (9x1), containing the following signals: - Position (x,y,z) [m] - Velocity (vx,vy,vz) [m/s] - Angles (Roll, Pitch, Yaw) [rad] The Actor state is defined in the global axis system. The state is superponed on the Initial position defined in the GUI. For more information, please click Help.
      settings: OpenFcn=open_system([gcb '/Actuator'],'mask')
      mask Help: eval('openHelp(222)')
      mask Display: image(imread('State.png'))
  STATE_Sphere_76_bus : Subsystem  Tag=actuator/StatePort  Priority=0  LoadFcn=load('PreScanStateActuatorData.mat')  mask(PreScan Sink Block: State){}
      mask help: The Actor State contains a vector signal of size (9x1), containing the following signals: - Position (x,y,z) [m] - Velocity (vx,vy,vz) [m/s] - Angles (Roll, Pitch, Yaw) [rad] The Actor state is defined in the global axis system. The state is superponed on the Initial position defined in the GUI. For more information, please click Help.
      settings: OpenFcn=open_system([gcb '/Actuator'],'mask')
      mask Help: eval('openHelp(222)')
      mask Display: image(imread('State.png'))
  STATE_Sphere_77_bus : Subsystem  Tag=actuator/StatePort  Priority=0  LoadFcn=load('PreScanStateActuatorData.mat')  mask(PreScan Sink Block: State){}
      mask help: The Actor State contains a vector signal of size (9x1), containing the following signals: - Position (x,y,z) [m] - Velocity (vx,vy,vz) [m/s] - Angles (Roll, Pitch, Yaw) [rad] The Actor state is defined in the global axis system. The state is superponed on the Initial position defined in the GUI. For more information, please click Help.
      settings: OpenFcn=open_system([gcb '/Actuator'],'mask')
      mask Help: eval('openHelp(222)')
      mask Display: image(imread('State.png'))
  STATE_Sphere_78_bus : Subsystem  Tag=actuator/StatePort  Priority=0  LoadFcn=load('PreScanStateActuatorData.mat')  mask(PreScan Sink Block: State){}
      mask help: The Actor State contains a vector signal of size (9x1), containing the following signals: - Position (x,y,z) [m] - Velocity (vx,vy,vz) [m/s] - Angles (Roll, Pitch, Yaw) [rad] The Actor state is defined in the global axis system. The state is superponed on the Initial position defined in the GUI. For more information, please click Help.
      settings: OpenFcn=open_system([gcb '/Actuator'],'mask')
      mask Help: eval('openHelp(222)')
      mask Display: image(imread('State.png'))
  STATE_Sphere_79_bus : Subsystem  Tag=actuator/StatePort  Priority=0  LoadFcn=load('PreScanStateActuatorData.mat')  mask(PreScan Sink Block: State){}
      mask help: The Actor State contains a vector signal of size (9x1), containing the following signals: - Position (x,y,z) [m] - Velocity (vx,vy,vz) [m/s] - Angles (Roll, Pitch, Yaw) [rad] The Actor state is defined in the global axis system. The state is superponed on the Initial position defined in the GUI. For more information, please click Help.
      settings: OpenFcn=open_system([gcb '/Actuator'],'mask')
      mask Help: eval('openHelp(222)')
      mask Display: image(imread('State.png'))
  STATE_Sphere_7_bus : Subsystem  Tag=actuator/StatePort  Priority=0  LoadFcn=load('PreScanStateActuatorData.mat')  mask(PreScan Sink Block: State){}
      mask help: The Actor State contains a vector signal of size (9x1), containing the following signals: - Position (x,y,z) [m] - Velocity (vx,vy,vz) [m/s] - Angles (Roll, Pitch, Yaw) [rad] The Actor state is defined in the global axis system. The state is superponed on the Initial position defined in the GUI. For more information, please click Help.
      settings: OpenFcn=open_system([gcb '/Actuator'],'mask')
      mask Help: eval('openHelp(222)')
      mask Display: image(imread('State.png'))
  STATE_Sphere_80_bus : Subsystem  Tag=actuator/StatePort  Priority=0  LoadFcn=load('PreScanStateActuatorData.mat')  mask(PreScan Sink Block: State){}
      mask help: The Actor State contains a vector signal of size (9x1), containing the following signals: - Position (x,y,z) [m] - Velocity (vx,vy,vz) [m/s] - Angles (Roll, Pitch, Yaw) [rad] The Actor state is defined in the global axis system. The state is superponed on the Initial position defined in the GUI. For more information, please click Help.
      settings: OpenFcn=open_system([gcb '/Actuator'],'mask')
      mask Help: eval('openHelp(222)')
      mask Display: image(imread('State.png'))
  STATE_Sphere_81_bus : Subsystem  Tag=actuator/StatePort  Priority=0  LoadFcn=load('PreScanStateActuatorData.mat')  mask(PreScan Sink Block: State){}
      mask help: The Actor State contains a vector signal of size (9x1), containing the following signals: - Position (x,y,z) [m] - Velocity (vx,vy,vz) [m/s] - Angles (Roll, Pitch, Yaw) [rad] The Actor state is defined in the global axis system. The state is superponed on the Initial position defined in the GUI. For more information, please click Help.
      settings: OpenFcn=open_system([gcb '/Actuator'],'mask')
      mask Help: eval('openHelp(222)')
      mask Display: image(imread('State.png'))
  STATE_Sphere_8_bus : Subsystem  Tag=actuator/StatePort  Priority=0  LoadFcn=load('PreScanStateActuatorData.mat')  mask(PreScan Sink Block: State){}
      mask help: The Actor State contains a vector signal of size (9x1), containing the following signals: - Position (x,y,z) [m] - Velocity (vx,vy,vz) [m/s] - Angles (Roll, Pitch, Yaw) [rad] The Actor state is defined in the global axis system. The state is superponed on the Initial position defined in the GUI. For more information, please click Help.
      settings: OpenFcn=open_system([gcb '/Actuator'],'mask')
      mask Help: eval('openHelp(222)')
      mask Display: image(imread('State.png'))
  STATE_Sphere_9_bus : Subsystem  Tag=actuator/StatePort  Priority=0  LoadFcn=load('PreScanStateActuatorData.mat')  mask(PreScan Sink Block: State){}
      mask help: The Actor State contains a vector signal of size (9x1), containing the following signals: - Position (x,y,z) [m] - Velocity (vx,vy,vz) [m/s] - Angles (Roll, Pitch, Yaw) [rad] The Actor state is defined in the global axis system. The state is superponed on the Initial position defined in the GUI. For more information, please click Help.
      settings: OpenFcn=open_system([gcb '/Actuator'],'mask')
      mask Help: eval('openHelp(222)')
      mask Display: image(imread('State.png'))
  ScenarioEngine : Subsystem  Tag=PreScanOpenScenarioBlock  Priority=10  LoadFcn=load PrescanSynchronizeData  mask(PreScan Simulation Core Block){TimeStep=1/20}
      mask prompts: TimeStep "Timestep [s]"
      mask help: Please do not remove this block from the PreScan compilation sheet, as it contains essential configuration parameters for a PreScan simulation.
      settings: DeleteFcn=PreScanBlockDeleteFcn;
      mask Display: image(imread('prescanlogo.ico'))
  Sphere_1 : Subsystem  Tag=WorldObjectSubSystem  InitFcn=UniqueId = '1001';
      mask init:
      | imagePath=which('Sphere.jpg');
      mask Display: image(imread(imagePath));color('white');text(0, 0, ' ID=1001\n')
  Sphere_10 : Subsystem  Tag=WorldObjectSubSystem  InitFcn=UniqueId = '1010';
      mask init:
      | imagePath=which('Sphere.jpg');
      mask Display: image(imread(imagePath));color('white');text(0, 0, ' ID=1010\n')
  Sphere_11 : Subsystem  Tag=WorldObjectSubSystem  InitFcn=UniqueId = '1011';
      mask init:
      | imagePath=which('Sphere.jpg');
      mask Display: image(imread(imagePath));color('white');text(0, 0, ' ID=1011\n')
  Sphere_12 : Subsystem  Tag=WorldObjectSubSystem  InitFcn=UniqueId = '1012';
      mask init:
      | imagePath=which('Sphere.jpg');
      mask Display: image(imread(imagePath));color('white');text(0, 0, ' ID=1012\n')
  Sphere_13 : Subsystem  Tag=WorldObjectSubSystem  InitFcn=UniqueId = '1013';
      mask init:
      | imagePath=which('Sphere.jpg');
      mask Display: image(imread(imagePath));color('white');text(0, 0, ' ID=1013\n')
  Sphere_14 : Subsystem  Tag=WorldObjectSubSystem  InitFcn=UniqueId = '1014';
      mask init:
      | imagePath=which('Sphere.jpg');
      mask Display: image(imread(imagePath));color('white');text(0, 0, ' ID=1014\n')
  Sphere_15 : Subsystem  Tag=WorldObjectSubSystem  InitFcn=UniqueId = '1015';
      mask init:
      | imagePath=which('Sphere.jpg');
      mask Display: image(imread(imagePath));color('white');text(0, 0, ' ID=1015\n')
  Sphere_16 : Subsystem  Tag=WorldObjectSubSystem  InitFcn=UniqueId = '1016';
      mask init:
      | imagePath=which('Sphere.jpg');
      mask Display: image(imread(imagePath));color('white');text(0, 0, ' ID=1016\n')
  Sphere_17 : Subsystem  Tag=WorldObjectSubSystem  InitFcn=UniqueId = '1017';
      mask init:
      | imagePath=which('Sphere.jpg');
      mask Display: image(imread(imagePath));color('white');text(0, 0, ' ID=1017\n')
  Sphere_18 : Subsystem  Tag=WorldObjectSubSystem  InitFcn=UniqueId = '1018';
      mask init:
      | imagePath=which('Sphere.jpg');
      mask Display: image(imread(imagePath));color('white');text(0, 0, ' ID=1018\n')
  Sphere_19 : Subsystem  Tag=WorldObjectSubSystem  InitFcn=UniqueId = '1019';
      mask init:
      | imagePath=which('Sphere.jpg');
      mask Display: image(imread(imagePath));color('white');text(0, 0, ' ID=1019\n')
  Sphere_2 : Subsystem  Tag=WorldObjectSubSystem  InitFcn=UniqueId = '1002';
      mask init:
      | imagePath=which('Sphere.jpg');
      mask Display: image(imread(imagePath));color('white');text(0, 0, ' ID=1002\n')
  Sphere_20 : Subsystem  Tag=WorldObjectSubSystem  InitFcn=UniqueId = '1020';
      mask init:
      | imagePath=which('Sphere.jpg');
      mask Display: image(imread(imagePath));color('white');text(0, 0, ' ID=1020\n')
  Sphere_21 : Subsystem  Tag=WorldObjectSubSystem  InitFcn=UniqueId = '1021';
      mask init:
      | imagePath=which('Sphere.jpg');
      mask Display: image(imread(imagePath));color('white');text(0, 0, ' ID=1021\n')
  Sphere_22 : Subsystem  Tag=WorldObjectSubSystem  InitFcn=UniqueId = '1022';
      mask init:
      | imagePath=which('Sphere.jpg');
      mask Display: image(imread(imagePath));color('white');text(0, 0, ' ID=1022\n')
  Sphere_23 : Subsystem  Tag=WorldObjectSubSystem  InitFcn=UniqueId = '1023';
      mask init:
      | imagePath=which('Sphere.jpg');
      mask Display: image(imread(imagePath));color('white');text(0, 0, ' ID=1023\n')
  Sphere_24 : Subsystem  Tag=WorldObjectSubSystem  InitFcn=UniqueId = '1024';
      mask init:
      | imagePath=which('Sphere.jpg');
      mask Display: image(imread(imagePath));color('white');text(0, 0, ' ID=1024\n')
  Sphere_25 : Subsystem  Tag=WorldObjectSubSystem  InitFcn=UniqueId = '1025';
      mask init:
      | imagePath=which('Sphere.jpg');
      mask Display: image(imread(imagePath));color('white');text(0, 0, ' ID=1025\n')
  Sphere_26 : Subsystem  Tag=WorldObjectSubSystem  InitFcn=UniqueId = '1026';
      mask init:
      | imagePath=which('Sphere.jpg');
      mask Display: image(imread(imagePath));color('white');text(0, 0, ' ID=1026\n')
  Sphere_27 : Subsystem  Tag=WorldObjectSubSystem  InitFcn=UniqueId = '1027';
      mask init:
      | imagePath=which('Sphere.jpg');
      mask Display: image(imread(imagePath));color('white');text(0, 0, ' ID=1027\n')
  Sphere_28 : Subsystem  Tag=WorldObjectSubSystem  InitFcn=UniqueId = '1028';
      mask init:
      | imagePath=which('Sphere.jpg');
      mask Display: image(imread(imagePath));color('white');text(0, 0, ' ID=1028\n')
  Sphere_29 : Subsystem  Tag=WorldObjectSubSystem  InitFcn=UniqueId = '1029';
      mask init:
      | imagePath=which('Sphere.jpg');
      mask Display: image(imread(imagePath));color('white');text(0, 0, ' ID=1029\n')
  Sphere_3 : Subsystem  Tag=WorldObjectSubSystem  InitFcn=UniqueId = '1003';
      mask init:
      | imagePath=which('Sphere.jpg');
      mask Display: image(imread(imagePath));color('white');text(0, 0, ' ID=1003\n')
  Sphere_30 : Subsystem  Tag=WorldObjectSubSystem  InitFcn=UniqueId = '1030';
      mask init:
      | imagePath=which('Sphere.jpg');
      mask Display: image(imread(imagePath));color('white');text(0, 0, ' ID=1030\n')
  Sphere_31 : Subsystem  Tag=WorldObjectSubSystem  InitFcn=UniqueId = '1031';
      mask init:
      | imagePath=which('Sphere.jpg');
      mask Display: image(imread(imagePath));color('white');text(0, 0, ' ID=1031\n')
  Sphere_32 : Subsystem  Tag=WorldObjectSubSystem  InitFcn=UniqueId = '1032';
      mask init:
      | imagePath=which('Sphere.jpg');
      mask Display: image(imread(imagePath));color('white');text(0, 0, ' ID=1032\n')
  Sphere_33 : Subsystem  Tag=WorldObjectSubSystem  InitFcn=UniqueId = '1033';
      mask init:
      | imagePath=which('Sphere.jpg');
      mask Display: image(imread(imagePath));color('white');text(0, 0, ' ID=1033\n')
  Sphere_34 : Subsystem  Tag=WorldObjectSubSystem  InitFcn=UniqueId = '1034';
      mask init:
      | imagePath=which('Sphere.jpg');
      mask Display: image(imread(imagePath));color('white');text(0, 0, ' ID=1034\n')
  Sphere_35 : Subsystem  Tag=WorldObjectSubSystem  InitFcn=UniqueId = '1035';
      mask init:
      | imagePath=which('Sphere.jpg');
      mask Display: image(imread(imagePath));color('white');text(0, 0, ' ID=1035\n')
  Sphere_36 : Subsystem  Tag=WorldObjectSubSystem  InitFcn=UniqueId = '1036';
      mask init:
      | imagePath=which('Sphere.jpg');
      mask Display: image(imread(imagePath));color('white');text(0, 0, ' ID=1036\n')
  Sphere_37 : Subsystem  Tag=WorldObjectSubSystem  InitFcn=UniqueId = '1037';
      mask init:
      | imagePath=which('Sphere.jpg');
      mask Display: image(imread(imagePath));color('white');text(0, 0, ' ID=1037\n')
  Sphere_38 : Subsystem  Tag=WorldObjectSubSystem  InitFcn=UniqueId = '1038';
      mask init:
      | imagePath=which('Sphere.jpg');
      mask Display: image(imread(imagePath));color('white');text(0, 0, ' ID=1038\n')
  Sphere_39 : Subsystem  Tag=WorldObjectSubSystem  InitFcn=UniqueId = '1039';
      mask init:
      | imagePath=which('Sphere.jpg');
      mask Display: image(imread(imagePath));color('white');text(0, 0, ' ID=1039\n')
  Sphere_4 : Subsystem  Tag=WorldObjectSubSystem  InitFcn=UniqueId = '1004';
      mask init:
      | imagePath=which('Sphere.jpg');
      mask Display: image(imread(imagePath));color('white');text(0, 0, ' ID=1004\n')
  Sphere_40 : Subsystem  Tag=WorldObjectSubSystem  InitFcn=UniqueId = '1040';
      mask init:
      | imagePath=which('Sphere.jpg');
      mask Display: image(imread(imagePath));color('white');text(0, 0, ' ID=1040\n')
  Sphere_41 : Subsystem  Tag=WorldObjectSubSystem  InitFcn=UniqueId = '1041';
      mask init:
      | imagePath=which('Sphere.jpg');
      mask Display: image(imread(imagePath));color('white');text(0, 0, ' ID=1041\n')
  Sphere_42 : Subsystem  Tag=WorldObjectSubSystem  InitFcn=UniqueId = '1042';
      mask init:
      | imagePath=which('Sphere.jpg');
      mask Display: image(imread(imagePath));color('white');text(0, 0, ' ID=1042\n')
  Sphere_43 : Subsystem  Tag=WorldObjectSubSystem  InitFcn=UniqueId = '1043';
      mask init:
      | imagePath=which('Sphere.jpg');
      mask Display: image(imread(imagePath));color('white');text(0, 0, ' ID=1043\n')
  Sphere_44 : Subsystem  Tag=WorldObjectSubSystem  InitFcn=UniqueId = '1044';
      mask init:
      | imagePath=which('Sphere.jpg');
      mask Display: image(imread(imagePath));color('white');text(0, 0, ' ID=1044\n')
  Sphere_45 : Subsystem  Tag=WorldObjectSubSystem  InitFcn=UniqueId = '1045';
      mask init:
      | imagePath=which('Sphere.jpg');
      mask Display: image(imread(imagePath));color('white');text(0, 0, ' ID=1045\n')
  Sphere_46 : Subsystem  Tag=WorldObjectSubSystem  InitFcn=UniqueId = '1046';
      mask init:
      | imagePath=which('Sphere.jpg');
      mask Display: image(imread(imagePath));color('white');text(0, 0, ' ID=1046\n')
  Sphere_47 : Subsystem  Tag=WorldObjectSubSystem  InitFcn=UniqueId = '1047';
      mask init:
      | imagePath=which('Sphere.jpg');
      mask Display: image(imread(imagePath));color('white');text(0, 0, ' ID=1047\n')
  Sphere_48 : Subsystem  Tag=WorldObjectSubSystem  InitFcn=UniqueId = '1048';
      mask init:
      | imagePath=which('Sphere.jpg');
      mask Display: image(imread(imagePath));color('white');text(0, 0, ' ID=1048\n')
  Sphere_49 : Subsystem  Tag=WorldObjectSubSystem  InitFcn=UniqueId = '1049';
      mask init:
      | imagePath=which('Sphere.jpg');
      mask Display: image(imread(imagePath));color('white');text(0, 0, ' ID=1049\n')
  Sphere_5 : Subsystem  Tag=WorldObjectSubSystem  InitFcn=UniqueId = '1005';
      mask init:
      | imagePath=which('Sphere.jpg');
      mask Display: image(imread(imagePath));color('white');text(0, 0, ' ID=1005\n')
  Sphere_50 : Subsystem  Tag=WorldObjectSubSystem  InitFcn=UniqueId = '1050';
      mask init:
      | imagePath=which('Sphere.jpg');
      mask Display: image(imread(imagePath));color('white');text(0, 0, ' ID=1050\n')
  Sphere_51 : Subsystem  Tag=WorldObjectSubSystem  InitFcn=UniqueId = '1051';
      mask init:
      | imagePath=which('Sphere.jpg');
      mask Display: image(imread(imagePath));color('white');text(0, 0, ' ID=1051\n')
  Sphere_52 : Subsystem  Tag=WorldObjectSubSystem  InitFcn=UniqueId = '1052';
      mask init:
      | imagePath=which('Sphere.jpg');
      mask Display: image(imread(imagePath));color('white');text(0, 0, ' ID=1052\n')
  Sphere_53 : Subsystem  Tag=WorldObjectSubSystem  InitFcn=UniqueId = '1053';
      mask init:
      | imagePath=which('Sphere.jpg');
      mask Display: image(imread(imagePath));color('white');text(0, 0, ' ID=1053\n')
  Sphere_54 : Subsystem  Tag=WorldObjectSubSystem  InitFcn=UniqueId = '1054';
      mask init:
      | imagePath=which('Sphere.jpg');
      mask Display: image(imread(imagePath));color('white');text(0, 0, ' ID=1054\n')
  Sphere_55 : Subsystem  Tag=WorldObjectSubSystem  InitFcn=UniqueId = '1055';
      mask init:
      | imagePath=which('Sphere.jpg');
      mask Display: image(imread(imagePath));color('white');text(0, 0, ' ID=1055\n')
  Sphere_56 : Subsystem  Tag=WorldObjectSubSystem  InitFcn=UniqueId = '1056';
      mask init:
      | imagePath=which('Sphere.jpg');
      mask Display: image(imread(imagePath));color('white');text(0, 0, ' ID=1056\n')
  Sphere_57 : Subsystem  Tag=WorldObjectSubSystem  InitFcn=UniqueId = '1057';
      mask init:
      | imagePath=which('Sphere.jpg');
      mask Display: image(imread(imagePath));color('white');text(0, 0, ' ID=1057\n')
  Sphere_58 : Subsystem  Tag=WorldObjectSubSystem  InitFcn=UniqueId = '1058';
      mask init:
      | imagePath=which('Sphere.jpg');
      mask Display: image(imread(imagePath));color('white');text(0, 0, ' ID=1058\n')
  Sphere_59 : Subsystem  Tag=WorldObjectSubSystem  InitFcn=UniqueId = '1059';
      mask init:
      | imagePath=which('Sphere.jpg');
      mask Display: image(imread(imagePath));color('white');text(0, 0, ' ID=1059\n')
  Sphere_6 : Subsystem  Tag=WorldObjectSubSystem  InitFcn=UniqueId = '1006';
      mask init:
      | imagePath=which('Sphere.jpg');
      mask Display: image(imread(imagePath));color('white');text(0, 0, ' ID=1006\n')
  Sphere_60 : Subsystem  Tag=WorldObjectSubSystem  InitFcn=UniqueId = '1060';
      mask init:
      | imagePath=which('Sphere.jpg');
      mask Display: image(imread(imagePath));color('white');text(0, 0, ' ID=1060\n')
  Sphere_61 : Subsystem  Tag=WorldObjectSubSystem  InitFcn=UniqueId = '1061';
      mask init:
      | imagePath=which('Sphere.jpg');
      mask Display: image(imread(imagePath));color('white');text(0, 0, ' ID=1061\n')
  Sphere_62 : Subsystem  Tag=WorldObjectSubSystem  InitFcn=UniqueId = '1062';
      mask init:
      | imagePath=which('Sphere.jpg');
      mask Display: image(imread(imagePath));color('white');text(0, 0, ' ID=1062\n')
  Sphere_63 : Subsystem  Tag=WorldObjectSubSystem  InitFcn=UniqueId = '1063';
      mask init:
      | imagePath=which('Sphere.jpg');
      mask Display: image(imread(imagePath));color('white');text(0, 0, ' ID=1063\n')
  Sphere_64 : Subsystem  Tag=WorldObjectSubSystem  InitFcn=UniqueId = '1064';
      mask init:
      | imagePath=which('Sphere.jpg');
      mask Display: image(imread(imagePath));color('white');text(0, 0, ' ID=1064\n')
  Sphere_65 : Subsystem  Tag=WorldObjectSubSystem  InitFcn=UniqueId = '1065';
      mask init:
      | imagePath=which('Sphere.jpg');
      mask Display: image(imread(imagePath));color('white');text(0, 0, ' ID=1065\n')
  Sphere_66 : Subsystem  Tag=WorldObjectSubSystem  InitFcn=UniqueId = '1066';
      mask init:
      | imagePath=which('Sphere.jpg');
      mask Display: image(imread(imagePath));color('white');text(0, 0, ' ID=1066\n')
  Sphere_67 : Subsystem  Tag=WorldObjectSubSystem  InitFcn=UniqueId = '1067';
      mask init:
      | imagePath=which('Sphere.jpg');
      mask Display: image(imread(imagePath));color('white');text(0, 0, ' ID=1067\n')
  Sphere_68 : Subsystem  Tag=WorldObjectSubSystem  InitFcn=UniqueId = '1068';
      mask init:
      | imagePath=which('Sphere.jpg');
      mask Display: image(imread(imagePath));color('white');text(0, 0, ' ID=1068\n')
  Sphere_69 : Subsystem  Tag=WorldObjectSubSystem  InitFcn=UniqueId = '1069';
      mask init:
      | imagePath=which('Sphere.jpg');
      mask Display: image(imread(imagePath));color('white');text(0, 0, ' ID=1069\n')
  Sphere_7 : Subsystem  Tag=WorldObjectSubSystem  InitFcn=UniqueId = '1007';
      mask init:
      | imagePath=which('Sphere.jpg');
      mask Display: image(imread(imagePath));color('white');text(0, 0, ' ID=1007\n')
  Sphere_70 : Subsystem  Tag=WorldObjectSubSystem  InitFcn=UniqueId = '1070';
      mask init:
      | imagePath=which('Sphere.jpg');
      mask Display: image(imread(imagePath));color('white');text(0, 0, ' ID=1070\n')
  Sphere_71 : Subsystem  Tag=WorldObjectSubSystem  InitFcn=UniqueId = '1071';
      mask init:
      | imagePath=which('Sphere.jpg');
      mask Display: image(imread(imagePath));color('white');text(0, 0, ' ID=1071\n')
  Sphere_72 : Subsystem  Tag=WorldObjectSubSystem  InitFcn=UniqueId = '1072';
      mask init:
      | imagePath=which('Sphere.jpg');
      mask Display: image(imread(imagePath));color('white');text(0, 0, ' ID=1072\n')
  Sphere_73 : Subsystem  Tag=WorldObjectSubSystem  InitFcn=UniqueId = '1073';
      mask init:
      | imagePath=which('Sphere.jpg');
      mask Display: image(imread(imagePath));color('white');text(0, 0, ' ID=1073\n')
  Sphere_74 : Subsystem  Tag=WorldObjectSubSystem  InitFcn=UniqueId = '1074';
      mask init:
      | imagePath=which('Sphere.jpg');
      mask Display: image(imread(imagePath));color('white');text(0, 0, ' ID=1074\n')
  Sphere_75 : Subsystem  Tag=WorldObjectSubSystem  InitFcn=UniqueId = '1075';
      mask init:
      | imagePath=which('Sphere.jpg');
      mask Display: image(imread(imagePath));color('white');text(0, 0, ' ID=1075\n')
  Sphere_76 : Subsystem  Tag=WorldObjectSubSystem  InitFcn=UniqueId = '1076';
      mask init:
      | imagePath=which('Sphere.jpg');
      mask Display: image(imread(imagePath));color('white');text(0, 0, ' ID=1076\n')
  Sphere_77 : Subsystem  Tag=WorldObjectSubSystem  InitFcn=UniqueId = '1077';
      mask init:
      | imagePath=which('Sphere.jpg');
      mask Display: image(imread(imagePath));color('white');text(0, 0, ' ID=1077\n')
  Sphere_78 : Subsystem  Tag=WorldObjectSubSystem  InitFcn=UniqueId = '1078';
      mask init:
      | imagePath=which('Sphere.jpg');
      mask Display: image(imread(imagePath));color('white');text(0, 0, ' ID=1078\n')
  Sphere_79 : Subsystem  Tag=WorldObjectSubSystem  InitFcn=UniqueId = '1079';
      mask init:
      | imagePath=which('Sphere.jpg');
      mask Display: image(imread(imagePath));color('white');text(0, 0, ' ID=1079\n')
  Sphere_8 : Subsystem  Tag=WorldObjectSubSystem  InitFcn=UniqueId = '1008';
      mask init:
      | imagePath=which('Sphere.jpg');
      mask Display: image(imread(imagePath));color('white');text(0, 0, ' ID=1008\n')
  Sphere_80 : Subsystem  Tag=WorldObjectSubSystem  InitFcn=UniqueId = '1080';
      mask init:
      | imagePath=which('Sphere.jpg');
      mask Display: image(imread(imagePath));color('white');text(0, 0, ' ID=1080\n')
  Sphere_81 : Subsystem  Tag=WorldObjectSubSystem  InitFcn=UniqueId = '1081';
      mask init:
      | imagePath=which('Sphere.jpg');
      mask Display: image(imread(imagePath));color('white');text(0, 0, ' ID=1081\n')
  Sphere_9 : Subsystem  Tag=WorldObjectSubSystem  InitFcn=UniqueId = '1009';
      mask init:
      | imagePath=which('Sphere.jpg');
      mask Display: image(imread(imagePath));color('white');text(0, 0, ' ID=1009\n')
  Synchronizer : Subsystem  Tag=PreScanSynchronizer  Priority=20  LoadFcn=load PrescanSynchronizeData  mask(PreScan Simulation Core Block){TimeStep=1/20}
      mask prompts: TimeStep "Timestep [s]"
      mask help: Please do not remove this block from the PreScan compilation sheet, as it contains essential configuration parameters for a PreScan simulation.
      settings: DeleteFcn=PreScanBlockDeleteFcn;
      mask Display: image(imread('prescanlogo.ico'))
  TIS_1 : Subsystem  Tag=sensor/TIS  Priority=30  LoadFcn=load('PrescanScannerSensorData.mat');load('PrescanScannerSensorMessage.mat')  mask(PreScan Source Block: Technology Independent Sensor (TIS)){}
      mask help: The Technology Independent Sensor (TIS) provides a sensor with all sensor-related influence factors (like noise, drift and accuracy) without being technology specific (like radar and lidar). The TIS detects the closest point on the geometry of an object. For more information, please click Help.
      settings: OpenFcn=open_system([gcb '/Sensor'],'mask')
      mask Help: eval('openHelp(449)')
      mask Display: image(imread('TIS.png'))
  wires:
  Sphere_1/1(STATE_Sphere_1_bus) -> STATE_Sphere_1_bus/1(STATE_Sphere_1_bus)
  SELF_Sphere_1/1(SELF_Sphere_1) -> Sphere_1/1(SELF_Sphere_1)
  Sphere_2/1(STATE_Sphere_2_bus) -> STATE_Sphere_2_bus/1(STATE_Sphere_2_bus)
  SELF_Sphere_2/1(SELF_Sphere_2) -> Sphere_2/1(SELF_Sphere_2)
  Sphere_3/1(STATE_Sphere_3_bus) -> STATE_Sphere_3_bus/1(STATE_Sphere_3_bus)
  SELF_Sphere_3/1(SELF_Sphere_3) -> Sphere_3/1(SELF_Sphere_3)
  Sphere_4/1(STATE_Sphere_4_bus) -> STATE_Sphere_4_bus/1(STATE_Sphere_4_bus)
  SELF_Sphere_4/1(SELF_Sphere_4) -> Sphere_4/1(SELF_Sphere_4)
  Sphere_5/1(STATE_Sphere_5_bus) -> STATE_Sphere_5_bus/1(STATE_Sphere_5_bus)
  SELF_Sphere_5/1(SELF_Sphere_5) -> Sphere_5/1(SELF_Sphere_5)
  Sphere_6/1(STATE_Sphere_6_bus) -> STATE_Sphere_6_bus/1(STATE_Sphere_6_bus)
  SELF_Sphere_6/1(SELF_Sphere_6) -> Sphere_6/1(SELF_Sphere_6)
  Sphere_7/1(STATE_Sphere_7_bus) -> STATE_Sphere_7_bus/1(STATE_Sphere_7_bus)
  SELF_Sphere_7/1(SELF_Sphere_7) -> Sphere_7/1(SELF_Sphere_7)
  Sphere_8/1(STATE_Sphere_8_bus) -> STATE_Sphere_8_bus/1(STATE_Sphere_8_bus)
  SELF_Sphere_8/1(SELF_Sphere_8) -> Sphere_8/1(SELF_Sphere_8)
  Sphere_9/1(STATE_Sphere_9_bus) -> STATE_Sphere_9_bus/1(STATE_Sphere_9_bus)
  SELF_Sphere_9/1(SELF_Sphere_9) -> Sphere_9/1(SELF_Sphere_9)
  Sphere_10/1(STATE_Sphere_10_bus) -> STATE_Sphere_10_bus/1(STATE_Sphere_10_bus)
  SELF_Sphere_10/1(SELF_Sphere_10) -> Sphere_10/1(SELF_Sphere_10)
  Sphere_11/1(STATE_Sphere_11_bus) -> STATE_Sphere_11_bus/1(STATE_Sphere_11_bus)
  SELF_Sphere_11/1(SELF_Sphere_11) -> Sphere_11/1(SELF_Sphere_11)
  Sphere_12/1(STATE_Sphere_12_bus) -> STATE_Sphere_12_bus/1(STATE_Sphere_12_bus)
  SELF_Sphere_12/1(SELF_Sphere_12) -> Sphere_12/1(SELF_Sphere_12)
  Sphere_13/1(STATE_Sphere_13_bus) -> STATE_Sphere_13_bus/1(STATE_Sphere_13_bus)
  SELF_Sphere_13/1(SELF_Sphere_13) -> Sphere_13/1(SELF_Sphere_13)
  Sphere_14/1(STATE_Sphere_14_bus) -> STATE_Sphere_14_bus/1(STATE_Sphere_14_bus)
  SELF_Sphere_14/1(SELF_Sphere_14) -> Sphere_14/1(SELF_Sphere_14)
  Sphere_15/1(STATE_Sphere_15_bus) -> STATE_Sphere_15_bus/1(STATE_Sphere_15_bus)
  SELF_Sphere_15/1(SELF_Sphere_15) -> Sphere_15/1(SELF_Sphere_15)
  Sphere_16/1(STATE_Sphere_16_bus) -> STATE_Sphere_16_bus/1(STATE_Sphere_16_bus)
  SELF_Sphere_16/1(SELF_Sphere_16) -> Sphere_16/1(SELF_Sphere_16)
  Sphere_17/1(STATE_Sphere_17_bus) -> STATE_Sphere_17_bus/1(STATE_Sphere_17_bus)
  SELF_Sphere_17/1(SELF_Sphere_17) -> Sphere_17/1(SELF_Sphere_17)
  Sphere_18/1(STATE_Sphere_18_bus) -> STATE_Sphere_18_bus/1(STATE_Sphere_18_bus)
  SELF_Sphere_18/1(SELF_Sphere_18) -> Sphere_18/1(SELF_Sphere_18)
  Sphere_19/1(STATE_Sphere_19_bus) -> STATE_Sphere_19_bus/1(STATE_Sphere_19_bus)
  SELF_Sphere_19/1(SELF_Sphere_19) -> Sphere_19/1(SELF_Sphere_19)
  Sphere_20/1(STATE_Sphere_20_bus) -> STATE_Sphere_20_bus/1(STATE_Sphere_20_bus)
  SELF_Sphere_20/1(SELF_Sphere_20) -> Sphere_20/1(SELF_Sphere_20)
  Sphere_21/1(STATE_Sphere_21_bus) -> STATE_Sphere_21_bus/1(STATE_Sphere_21_bus)
  SELF_Sphere_21/1(SELF_Sphere_21) -> Sphere_21/1(SELF_Sphere_21)
  Sphere_22/1(STATE_Sphere_22_bus) -> STATE_Sphere_22_bus/1(STATE_Sphere_22_bus)
  SELF_Sphere_22/1(SELF_Sphere_22) -> Sphere_22/1(SELF_Sphere_22)
  Sphere_23/1(STATE_Sphere_23_bus) -> STATE_Sphere_23_bus/1(STATE_Sphere_23_bus)
  SELF_Sphere_23/1(SELF_Sphere_23) -> Sphere_23/1(SELF_Sphere_23)
  Sphere_24/1(STATE_Sphere_24_bus) -> STATE_Sphere_24_bus/1(STATE_Sphere_24_bus)
  SELF_Sphere_24/1(SELF_Sphere_24) -> Sphere_24/1(SELF_Sphere_24)
  Sphere_25/1(STATE_Sphere_25_bus) -> STATE_Sphere_25_bus/1(STATE_Sphere_25_bus)
  SELF_Sphere_25/1(SELF_Sphere_25) -> Sphere_25/1(SELF_Sphere_25)
  Sphere_26/1(STATE_Sphere_26_bus) -> STATE_Sphere_26_bus/1(STATE_Sphere_26_bus)
  SELF_Sphere_26/1(SELF_Sphere_26) -> Sphere_26/1(SELF_Sphere_26)
  Sphere_27/1(STATE_Sphere_27_bus) -> STATE_Sphere_27_bus/1(STATE_Sphere_27_bus)
  SELF_Sphere_27/1(SELF_Sphere_27) -> Sphere_27/1(SELF_Sphere_27)
  Sphere_28/1(STATE_Sphere_28_bus) -> STATE_Sphere_28_bus/1(STATE_Sphere_28_bus)
  SELF_Sphere_28/1(SELF_Sphere_28) -> Sphere_28/1(SELF_Sphere_28)
  Sphere_29/1(STATE_Sphere_29_bus) -> STATE_Sphere_29_bus/1(STATE_Sphere_29_bus)
  SELF_Sphere_29/1(SELF_Sphere_29) -> Sphere_29/1(SELF_Sphere_29)
  Sphere_30/1(STATE_Sphere_30_bus) -> STATE_Sphere_30_bus/1(STATE_Sphere_30_bus)
  SELF_Sphere_30/1(SELF_Sphere_30) -> Sphere_30/1(SELF_Sphere_30)
  Sphere_31/1(STATE_Sphere_31_bus) -> STATE_Sphere_31_bus/1(STATE_Sphere_31_bus)
  SELF_Sphere_31/1(SELF_Sphere_31) -> Sphere_31/1(SELF_Sphere_31)
  Sphere_32/1(STATE_Sphere_32_bus) -> STATE_Sphere_32_bus/1(STATE_Sphere_32_bus)
  SELF_Sphere_32/1(SELF_Sphere_32) -> Sphere_32/1(SELF_Sphere_32)
  Sphere_33/1(STATE_Sphere_33_bus) -> STATE_Sphere_33_bus/1(STATE_Sphere_33_bus)
  SELF_Sphere_33/1(SELF_Sphere_33) -> Sphere_33/1(SELF_Sphere_33)
  Sphere_34/1(STATE_Sphere_34_bus) -> STATE_Sphere_34_bus/1(STATE_Sphere_34_bus)
  SELF_Sphere_34/1(SELF_Sphere_34) -> Sphere_34/1(SELF_Sphere_34)
  Sphere_35/1(STATE_Sphere_35_bus) -> STATE_Sphere_35_bus/1(STATE_Sphere_35_bus)
  SELF_Sphere_35/1(SELF_Sphere_35) -> Sphere_35/1(SELF_Sphere_35)
  Sphere_36/1(STATE_Sphere_36_bus) -> STATE_Sphere_36_bus/1(STATE_Sphere_36_bus)
  SELF_Sphere_36/1(SELF_Sphere_36) -> Sphere_36/1(SELF_Sphere_36)
  Sphere_37/1(STATE_Sphere_37_bus) -> STATE_Sphere_37_bus/1(STATE_Sphere_37_bus)
  SELF_Sphere_37/1(SELF_Sphere_37) -> Sphere_37/1(SELF_Sphere_37)
  Sphere_38/1(STATE_Sphere_38_bus) -> STATE_Sphere_38_bus/1(STATE_Sphere_38_bus)
  SELF_Sphere_38/1(SELF_Sphere_38) -> Sphere_38/1(SELF_Sphere_38)
  Sphere_39/1(STATE_Sphere_39_bus) -> STATE_Sphere_39_bus/1(STATE_Sphere_39_bus)
  SELF_Sphere_39/1(SELF_Sphere_39) -> Sphere_39/1(SELF_Sphere_39)
  Sphere_40/1(STATE_Sphere_40_bus) -> STATE_Sphere_40_bus/1(STATE_Sphere_40_bus)
  SELF_Sphere_40/1(SELF_Sphere_40) -> Sphere_40/1(SELF_Sphere_40)
  Sphere_41/1(STATE_Sphere_41_bus) -> STATE_Sphere_41_bus/1(STATE_Sphere_41_bus)
  SELF_Sphere_41/1(SELF_Sphere_41) -> Sphere_41/1(SELF_Sphere_41)
  Sphere_42/1(STATE_Sphere_42_bus) -> STATE_Sphere_42_bus/1(STATE_Sphere_42_bus)
  SELF_Sphere_42/1(SELF_Sphere_42) -> Sphere_42/1(SELF_Sphere_42)
  Sphere_43/1(STATE_Sphere_43_bus) -> STATE_Sphere_43_bus/1(STATE_Sphere_43_bus)
  SELF_Sphere_43/1(SELF_Sphere_43) -> Sphere_43/1(SELF_Sphere_43)
  Sphere_44/1(STATE_Sphere_44_bus) -> STATE_Sphere_44_bus/1(STATE_Sphere_44_bus)
  SELF_Sphere_44/1(SELF_Sphere_44) -> Sphere_44/1(SELF_Sphere_44)
  Sphere_45/1(STATE_Sphere_45_bus) -> STATE_Sphere_45_bus/1(STATE_Sphere_45_bus)
  SELF_Sphere_45/1(SELF_Sphere_45) -> Sphere_45/1(SELF_Sphere_45)
  Sphere_46/1(STATE_Sphere_46_bus) -> STATE_Sphere_46_bus/1(STATE_Sphere_46_bus)
  SELF_Sphere_46/1(SELF_Sphere_46) -> Sphere_46/1(SELF_Sphere_46)
  Sphere_47/1(STATE_Sphere_47_bus) -> STATE_Sphere_47_bus/1(STATE_Sphere_47_bus)
  SELF_Sphere_47/1(SELF_Sphere_47) -> Sphere_47/1(SELF_Sphere_47)
  Sphere_48/1(STATE_Sphere_48_bus) -> STATE_Sphere_48_bus/1(STATE_Sphere_48_bus)
  SELF_Sphere_48/1(SELF_Sphere_48) -> Sphere_48/1(SELF_Sphere_48)
  Sphere_49/1(STATE_Sphere_49_bus) -> STATE_Sphere_49_bus/1(STATE_Sphere_49_bus)
  SELF_Sphere_49/1(SELF_Sphere_49) -> Sphere_49/1(SELF_Sphere_49)
  Sphere_50/1(STATE_Sphere_50_bus) -> STATE_Sphere_50_bus/1(STATE_Sphere_50_bus)
  SELF_Sphere_50/1(SELF_Sphere_50) -> Sphere_50/1(SELF_Sphere_50)
  Sphere_51/1(STATE_Sphere_51_bus) -> STATE_Sphere_51_bus/1(STATE_Sphere_51_bus)
  SELF_Sphere_51/1(SELF_Sphere_51) -> Sphere_51/1(SELF_Sphere_51)
  Sphere_52/1(STATE_Sphere_52_bus) -> STATE_Sphere_52_bus/1(STATE_Sphere_52_bus)
  SELF_Sphere_52/1(SELF_Sphere_52) -> Sphere_52/1(SELF_Sphere_52)
  Sphere_53/1(STATE_Sphere_53_bus) -> STATE_Sphere_53_bus/1(STATE_Sphere_53_bus)
  SELF_Sphere_53/1(SELF_Sphere_53) -> Sphere_53/1(SELF_Sphere_53)
  Sphere_54/1(STATE_Sphere_54_bus) -> STATE_Sphere_54_bus/1(STATE_Sphere_54_bus)
  SELF_Sphere_54/1(SELF_Sphere_54) -> Sphere_54/1(SELF_Sphere_54)
  Sphere_55/1(STATE_Sphere_55_bus) -> STATE_Sphere_55_bus/1(STATE_Sphere_55_bus)
  SELF_Sphere_55/1(SELF_Sphere_55) -> Sphere_55/1(SELF_Sphere_55)
  Sphere_56/1(STATE_Sphere_56_bus) -> STATE_Sphere_56_bus/1(STATE_Sphere_56_bus)
  SELF_Sphere_56/1(SELF_Sphere_56) -> Sphere_56/1(SELF_Sphere_56)
  Sphere_57/1(STATE_Sphere_57_bus) -> STATE_Sphere_57_bus/1(STATE_Sphere_57_bus)
  SELF_Sphere_57/1(SELF_Sphere_57) -> Sphere_57/1(SELF_Sphere_57)
  Sphere_58/1(STATE_Sphere_58_bus) -> STATE_Sphere_58_bus/1(STATE_Sphere_58_bus)
  SELF_Sphere_58/1(SELF_Sphere_58) -> Sphere_58/1(SELF_Sphere_58)
  Sphere_59/1(STATE_Sphere_59_bus) -> STATE_Sphere_59_bus/1(STATE_Sphere_59_bus)
  SELF_Sphere_59/1(SELF_Sphere_59) -> Sphere_59/1(SELF_Sphere_59)
  Sphere_60/1(STATE_Sphere_60_bus) -> STATE_Sphere_60_bus/1(STATE_Sphere_60_bus)
  SELF_Sphere_60/1(SELF_Sphere_60) -> Sphere_60/1(SELF_Sphere_60)
  Sphere_61/1(STATE_Sphere_61_bus) -> STATE_Sphere_61_bus/1(STATE_Sphere_61_bus)
  SELF_Sphere_61/1(SELF_Sphere_61) -> Sphere_61/1(SELF_Sphere_61)
  Sphere_62/1(STATE_Sphere_62_bus) -> STATE_Sphere_62_bus/1(STATE_Sphere_62_bus)
  SELF_Sphere_62/1(SELF_Sphere_62) -> Sphere_62/1(SELF_Sphere_62)
  Sphere_63/1(STATE_Sphere_63_bus) -> STATE_Sphere_63_bus/1(STATE_Sphere_63_bus)
  SELF_Sphere_63/1(SELF_Sphere_63) -> Sphere_63/1(SELF_Sphere_63)
  Sphere_64/1(STATE_Sphere_64_bus) -> STATE_Sphere_64_bus/1(STATE_Sphere_64_bus)
  SELF_Sphere_64/1(SELF_Sphere_64) -> Sphere_64/1(SELF_Sphere_64)
  Sphere_65/1(STATE_Sphere_65_bus) -> STATE_Sphere_65_bus/1(STATE_Sphere_65_bus)
  SELF_Sphere_65/1(SELF_Sphere_65) -> Sphere_65/1(SELF_Sphere_65)
  Sphere_66/1(STATE_Sphere_66_bus) -> STATE_Sphere_66_bus/1(STATE_Sphere_66_bus)
  SELF_Sphere_66/1(SELF_Sphere_66) -> Sphere_66/1(SELF_Sphere_66)
  Sphere_67/1(STATE_Sphere_67_bus) -> STATE_Sphere_67_bus/1(STATE_Sphere_67_bus)
  SELF_Sphere_67/1(SELF_Sphere_67) -> Sphere_67/1(SELF_Sphere_67)
  Sphere_68/1(STATE_Sphere_68_bus) -> STATE_Sphere_68_bus/1(STATE_Sphere_68_bus)
  SELF_Sphere_68/1(SELF_Sphere_68) -> Sphere_68/1(SELF_Sphere_68)
  Sphere_69/1(STATE_Sphere_69_bus) -> STATE_Sphere_69_bus/1(STATE_Sphere_69_bus)
  SELF_Sphere_69/1(SELF_Sphere_69) -> Sphere_69/1(SELF_Sphere_69)
  Sphere_70/1(STATE_Sphere_70_bus) -> STATE_Sphere_70_bus/1(STATE_Sphere_70_bus)
  SELF_Sphere_70/1(SELF_Sphere_70) -> Sphere_70/1(SELF_Sphere_70)
  Sphere_71/1(STATE_Sphere_71_bus) -> STATE_Sphere_71_bus/1(STATE_Sphere_71_bus)
  SELF_Sphere_71/1(SELF_Sphere_71) -> Sphere_71/1(SELF_Sphere_71)
  Sphere_72/1(STATE_Sphere_72_bus) -> STATE_Sphere_72_bus/1(STATE_Sphere_72_bus)
  SELF_Sphere_72/1(SELF_Sphere_72) -> Sphere_72/1(SELF_Sphere_72)
  Sphere_73/1(STATE_Sphere_73_bus) -> STATE_Sphere_73_bus/1(STATE_Sphere_73_bus)
  SELF_Sphere_73/1(SELF_Sphere_73) -> Sphere_73/1(SELF_Sphere_73)
  Sphere_74/1(STATE_Sphere_74_bus) -> STATE_Sphere_74_bus/1(STATE_Sphere_74_bus)
  SELF_Sphere_74/1(SELF_Sphere_74) -> Sphere_74/1(SELF_Sphere_74)
  Sphere_75/1(STATE_Sphere_75_bus) -> STATE_Sphere_75_bus/1(STATE_Sphere_75_bus)
  SELF_Sphere_75/1(SELF_Sphere_75) -> Sphere_75/1(SELF_Sphere_75)
  Sphere_76/1(STATE_Sphere_76_bus) -> STATE_Sphere_76_bus/1(STATE_Sphere_76_bus)
  SELF_Sphere_76/1(SELF_Sphere_76) -> Sphere_76/1(SELF_Sphere_76)
  Sphere_77/1(STATE_Sphere_77_bus) -> STATE_Sphere_77_bus/1(STATE_Sphere_77_bus)
  SELF_Sphere_77/1(SELF_Sphere_77) -> Sphere_77/1(SELF_Sphere_77)
  Sphere_78/1(STATE_Sphere_78_bus) -> STATE_Sphere_78_bus/1(STATE_Sphere_78_bus)
  SELF_Sphere_78/1(SELF_Sphere_78) -> Sphere_78/1(SELF_Sphere_78)
  Sphere_79/1(STATE_Sphere_79_bus) -> STATE_Sphere_79_bus/1(STATE_Sphere_79_bus)
  SELF_Sphere_79/1(SELF_Sphere_79) -> Sphere_79/1(SELF_Sphere_79)
  Sphere_80/1(STATE_Sphere_80_bus) -> STATE_Sphere_80_bus/1(STATE_Sphere_80_bus)
  SELF_Sphere_80/1(SELF_Sphere_80) -> Sphere_80/1(SELF_Sphere_80)
  Sphere_81/1(STATE_Sphere_81_bus) -> STATE_Sphere_81_bus/1(STATE_Sphere_81_bus)
  SELF_Sphere_81/1(SELF_Sphere_81) -> Sphere_81/1(SELF_Sphere_81)
  Cone_1/1(STATE_Cone_1_bus) -> STATE_Cone_1_bus/1(STATE_Cone_1_bus)
  SELF_Cone_1/1(SELF_Cone_1) -> Cone_1/1(SELF_Cone_1)
  TIS_1/1(TIS_1) -> Cone_1/2(TIS_1)
  Cylinder_1/1(STATE_Cylinder_1_bus) -> STATE_Cylinder_1_bus/1(STATE_Cylinder_1_bus)
  SELF_Cylinder_1/1(SELF_Cylinder_1) -> Cylinder_1/1(SELF_Cylinder_1)
  Cylinder_2/1(STATE_Cylinder_2_bus) -> STATE_Cylinder_2_bus/1(STATE_Cylinder_2_bus)
  SELF_Cylinder_2/1(SELF_Cylinder_2) -> Cylinder_2/1(SELF_Cylinder_2)
